simulink model "Copter_Plane_V10_sim_jy"  (R2021a)
settings: Solver=ode1  StartTime=0.0  StopTime=200  FixedStep=dt  RelTol=1e-3
undefined symbols (not defined in the file or in its folder): AC_Attitude, AC_PosControl, algo_accel_target_0, algo_accel_target_1, algo_accel_target_2, algo_arspeed, algo_attitude_target_euler_angle_0, algo_attitude_target_euler_angle_1, algo_attitude_target_euler_angle_2, algo_attitude_target_euler_rate_0, algo_attitude_target_euler_rate_1, algo_attitude_target_euler_rate_2, algo_climb_rate_cms, algo_curPathPoint_LLA_0, algo_curPathPoint_LLA_1, algo_curPosNED_0, algo_curPosNED_1, algo_curr_alt, algo_curr_pos_0, algo_curr_pos_1, algo_curr_vel_0, algo_curr_vel_1, algo_curr_vel_2, algo_current_loc_0, algo_current_loc_1, algo_curVelNED_0, algo_curVelNED_1, algo_flightControlMode, algo_flightTaskMode, algo_heightCmd_sl, algo_hgt_dem, algo_k_aileron, algo_k_elevator, algo_k_rudder, algo_k_throttle, algo_latAccDem, algo_limit_pos_up, algo_maxClimbSpeed, algo_mode, algo_nav_pitch_cd, algo_nav_roll, algo_pitch, algo_pitch_dem, algo_pitch_in, algo_pitch_target_pilot, algo_plane_mode, algo_pos_target_0, algo_pos_target_1, algo_pos_target_2, algo_prePathPoint_LLA_0, algo_prePathPoint_LLA_1, algo_pwm_out_1, algo_pwm_out_2, algo_pwm_out_3, algo_pwm_out_4, algo_rate_target_ang_vel_0, algo_rate_target_ang_vel_1, algo_rate_target_ang_vel_2, algo_remote_ct_st_pitch, algo_remote_ct_st_roll ... (+39)
libraries: aerolibasang x1, sharedtransform x1
(part 1 of 2)
settings Model: PauseTimes=6.8  Creator=a4327481  LastModifiedBy=a4327481
settings SolverCC: AlgebraicLoopSolver=TrustRegion
settings DebuggingCC: SFMachineParentedDataDiag=warning

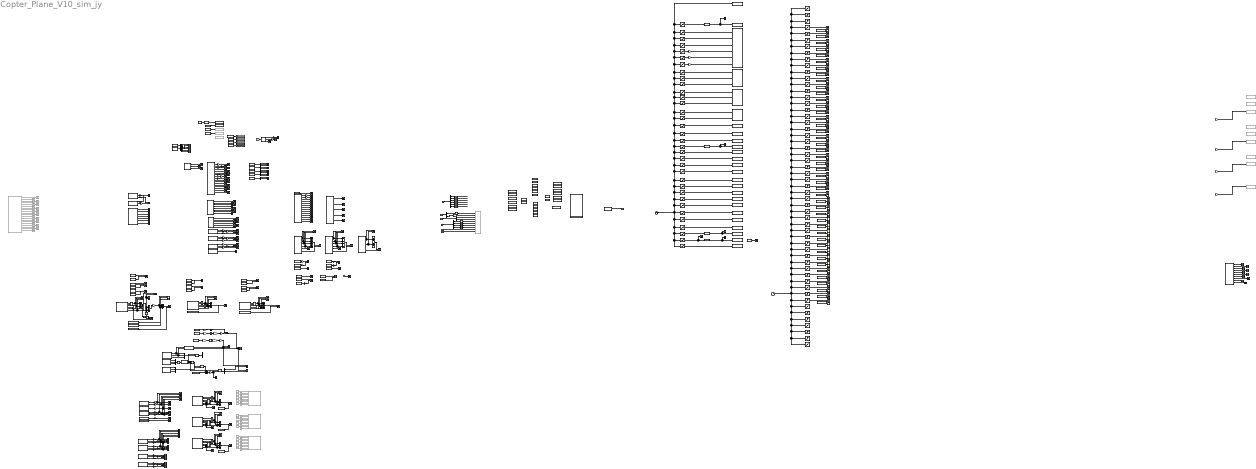
== system Copter_Plane_V10_sim_jy ==
  CTRL_wp : Inport
  PathModeOut : Inport  Port=2  OutDataTypeStr=Bus: BUS_TASK_PATH_OutParam
  TASK_COMMON_OutParam : Inport  Port=3  OutDataTypeStr=Bus: BUS_TASK_COMMON_OutParam
  NAVI2CONTROL : Inport  Port=4  OutDataTypeStr=Bus: BUS_TO_CONTROL
  EAS_Algo : Inport  Port=5  OutDataTypeStr=Bus: BUS_AIRSPEED
  IMU : Inport  Port=6  OutDataTypeStr=Bus: BUS_IMU
  AC_Attitude : DataStoreMemory  DataStoreName=AC_Attitude  ReadBeforeWriteMsg=warning  WriteAfterWriteMsg=warning  WriteAfterReadMsg=warning  InitialValue=AC_Attitude  ShowAdditionalParam=off  OutDataTypeStr=Bus: BUS_CTRL_AC_Attitude
  AC_PosControl : DataStoreMemory  DataStoreName=AC_PosControl  ReadBeforeWriteMsg=warning  WriteAfterWriteMsg=warning  WriteAfterReadMsg=warning  InitialValue=AC_PosControl  ShowAdditionalParam=off  OutDataTypeStr=Bus: BUS_CTRL_AC_PosControl
  AC_rate_pitch_pid : DataStoreMemory  DataStoreName=AC_rate_pitch_pid  ReadBeforeWriteMsg=warning  WriteAfterWriteMsg=warning  WriteAfterReadMsg=warning  InitialValue=AC_rate_pitch_pid  ShowAdditionalParam=off  OutDataTypeStr=Bus: BUS_CTRL_PID
  AC_rate_roll_pid : DataStoreMemory  DataStoreName=AC_rate_roll_pid  ReadBeforeWriteMsg=warning  WriteAfterWriteMsg=warning  WriteAfterReadMsg=warning  InitialValue=AC_rate_roll_pid  ShowAdditionalParam=off  OutDataTypeStr=Bus: BUS_CTRL_PID
  AC_rate_yaw_pid : DataStoreMemory  DataStoreName=AC_rate_yaw_pid  ReadBeforeWriteMsg=warning  WriteAfterWriteMsg=warning  WriteAfterReadMsg=warning  InitialValue=AC_rate_yaw_pid  ShowAdditionalParam=off  OutDataTypeStr=Bus: BUS_CTRL_PID
  AP_L1 : DataStoreMemory  DataStoreName=AP_L1  ReadBeforeWriteMsg=warning  WriteAfterWriteMsg=warning  WriteAfterReadMsg=warning  InitialValue=AP_L1  ShowAdditionalParam=off  OutDataTypeStr=Bus: BUS_CTRL_AP_L1
  AP_Motors : DataStoreMemory  DataStoreName=AP_Motors  ReadBeforeWriteMsg=warning  WriteAfterWriteMsg=warning  WriteAfterReadMsg=warning  InitialValue=AP_Motors  VectorParams1D=off  ShowAdditionalParam=off  OutDataTypeStr=Bus: BUS_CTRL_AP_Motors
  AP_TECS : DataStoreMemory  DataStoreName=AP_TECS  ReadBeforeWriteMsg=warning  WriteAfterWriteMsg=warning  WriteAfterReadMsg=warning  InitialValue=AP_TECS  ShowAdditionalParam=off  OutDataTypeStr=Bus: BUS_CTRL_AP_TECS
  AP_rate_pitch : DataStoreMemory  DataStoreName=AP_rate_pitch  ReadBeforeWriteMsg=warning  WriteAfterWriteMsg=warning  WriteAfterReadMsg=warning  InitialValue=AP_rate_pitch  ShowAdditionalParam=off  OutDataTypeStr=Bus: BUS_CTRL_AP_PID_pitch
  AP_rate_roll : DataStoreMemory  DataStoreName=AP_rate_roll  ReadBeforeWriteMsg=warning  WriteAfterWriteMsg=warning  WriteAfterReadMsg=warning  InitialValue=AP_rate_roll  ShowAdditionalParam=off  OutDataTypeStr=Bus: BUS_CTRL_AP_PID_roll
  AP_rate_yaw : DataStoreMemory  DataStoreName=AP_rate_yaw  ReadBeforeWriteMsg=warning  WriteAfterWriteMsg=warning  WriteAfterReadMsg=warning  InitialValue=AP_rate_yaw  ShowAdditionalParam=off  OutDataTypeStr=Bus: BUS_CTRL_AP_PID_yaw
  Add : Sum  Inputs=++++
  Add{4,6,10..13} (6 alike) : Sum  Inputs=+++
  Add14 : Sum  Inputs=++++
  Add{3,9,15..16} (4 alike) : Sum
  Bus Selector : BusSelector  OutputSignals=curVelNED,curLLA
  Bus Selector1 : BusSelector  OutputSignals=pitchd,rolld,yawd,alt
  Bus Selector2 : BusSelector  OutputSignals=gyro_x,gyro_y,gyro_z,accel_x,accel_y,accel_z
  Bus Selector3 : BusSelector  OutputSignals=airspeed_indicate,EAS2TAS_Algo
  Clock1 : Clock
  Clock2 : Clock
  Constant1 : Constant  Value=500/4500*0.95+0.05
  Constant10 : Constant  Value=500/4500*0.95+0.05
  Constant18 : Constant  Commented=on  Value=0.3
  Constant19 : Constant  Commented=on  Value=0.15
  Constant20 : Constant  Commented=on  Value=0.1
  Constant{21,26,33,38,43,48} (6 alike) : Constant  Commented=on  Value=0
  Constant22 : Constant  Commented=on  Value=0.25
  Constant{23..25,35..37,45..47} (9 alike) : Constant  Commented=on  Value=20
  Constant27 : Constant  Value=10  OutDataTypeStr=int16
  Constant28 : Constant  Commented=on
  Constant29 : Constant  Commented=on  Value=0.3
  Constant31 : Constant  Commented=on  Value=0.15
  Constant32 : Constant  Commented=on  Value=0.2
  Constant34 : Constant  Commented=on  Value=0.25
  Constant39 : Constant  Commented=on
  Constant40 : Constant  Commented=on  Value=0.3
  Constant41 : Constant  Commented=on  Value=0.15
  Constant42 : Constant  Commented=on  Value=0.1
  Constant44 : Constant  Commented=on  Value=0.25
  Constant49 : Constant  Commented=on
  Constant9 : Constant  Value=0.4
  Copter_Plane : DataStoreMemory  DataStoreName=Copter_Plane  ReadBeforeWriteMsg=warning  WriteAfterWriteMsg=warning  WriteAfterReadMsg=warning  InitialValue=Copter_Plane  VectorParams1D=off  ShowAdditionalParam=off  OutDataTypeStr=Bus: BUS_CTRL_Copter_Plane
  Curr_sate : DataStoreMemory  DataStoreName=Curr_sate  ReadBeforeWriteMsg=warning  WriteAfterWriteMsg=warning  WriteAfterReadMsg=warning  InitialValue=Curr_sate  VectorParams1D=off  ShowAdditionalParam=off  OutDataTypeStr=Bus: BUS_CTRL_Curr_sate
  Data Store Read : DataStoreRead  DataStoreName=SRV_Channel  IndexOptions=Index vector (dialog)  Indices=1  OutputSizes=1
  Data Store Read1 : DataStoreRead  DataStoreName=SINS  DataStoreElements=SINS.gyro_x#SINS.gyro_y#SINS.gyro_z#SINS.accel_x#SINS.accel_y#SINS.accel_z#SINS.roll#SINS.pitch#SINS.yaw#SINS.curr_vel(:,:)#SINS.curr_loc(:,:)#SINS.curr_alt#SINS.aspeed#SINS.EAS2TAS#SINS.groundspeed_vector(:,:)#SINS.curr_pos(:,:)#SINS.z_accel_meas  IndexOptions=Index vector (dialog)  Indices=1  OutputSizes=1
  Data Store Read10 : DataStoreRead  DataStoreName=AC_PosControl  DataStoreElements=AC_PosControl.vel_target(:,2)  IndexOptions=Index vector (dialog)  Indices=1  OutputSizes=1
  Data Store Read100 : DataStoreRead  DataStoreName=AP_rate_pitch  DataStoreElements=AP_rate_pitch.pid_info_P#AP_rate_pitch.pid_info_I#AP_rate_pitch.pid_info_D#AP_rate_pitch.pid_info_FF#AP_rate_pitch.pid_info_Dmod#AP_rate_pitch.last_out  IndexOptions=Index vector (dialog)  Indices=1  OutputSizes=1
  Data Store Read101 : DataStoreRead  DataStoreName=AP_rate_yaw  DataStoreElements=AP_rate_yaw.pid_info_I#AP_rate_yaw.pid_info_D#AP_rate_yaw.last_out  IndexOptions=Index vector (dialog)  Indices=1  OutputSizes=1
  Data Store Read105 : DataStoreRead  DataStoreName=AP_L1  DataStoreElements=AP_L1.L1_dist#AP_L1.last_Nu#AP_L1.latAccDem#AP_L1.nav_bearing#AP_L1.bearing_error  IndexOptions=Index vector (dialog)  Indices=1  OutputSizes=1
  Data Store Read107 : DataStoreRead  DataStoreName=AC_PosControl  DataStoreElements=AC_PosControl.accel_desired(:,:)  IndexOptions=Index vector (dialog)  Indices=1  OutputSizes=1
  Data Store Read108 : DataStoreRead  DataStoreName=AC_PosControl  DataStoreElements=AC_PosControl.accel_target(:,:)  IndexOptions=Index vector (dialog)  Indices=1  OutputSizes=1
  Data Store Read109 : DataStoreRead  DataStoreName=SINS  DataStoreElements=SINS.curr_vel(:,:)  IndexOptions=Index vector (dialog)  Indices=1  OutputSizes=1
  Data Store Read11 : DataStoreRead  DataStoreName=AC_PosControl  DataStoreElements=AC_PosControl.pos_target(:,2)  IndexOptions=Index vector (dialog)  Indices=1  OutputSizes=1
  Data Store Read112 : DataStoreRead  DataStoreName=AC_PosControl  DataStoreElements=AC_PosControl.vel_target(:,:)  IndexOptions=Index vector (dialog)  Indices=1  OutputSizes=1
  Data Store Read114 : DataStoreRead  DataStoreName=AC_PosControl  DataStoreElements=AC_PosControl.accel_target(:,3)  IndexOptions=Index vector (dialog)  Indices=1  OutputSizes=1
  Data Store Read116 : DataStoreRead  DataStoreName=SINS  DataStoreElements=SINS.z_accel_meas  IndexOptions=Index vector (dialog)  Indices=1  OutputSizes=1
  Data Store Read117 : DataStoreRead  DataStoreName=SINS  DataStoreElements=SINS.curr_vel(:,3)  IndexOptions=Index vector (dialog)  Indices=1  OutputSizes=1
  Data Store Read118 : DataStoreRead  DataStoreName=AC_PosControl  DataStoreElements=AC_PosControl.vel_desired(:,3)#AC_PosControl.vel_target(:,3)  IndexOptions=Index vector (dialog)  Indices=1  OutputSizes=1
  Data Store Read119 : DataStoreRead  DataStoreName=AC_PosControl  DataStoreElements=AC_PosControl.pos_target(:,3)  IndexOptions=Index vector (dialog)  Indices=1  OutputSizes=1
  Data Store Read12 : DataStoreRead  DataStoreName=AC_PosControl  DataStoreElements=AC_PosControl.pos_target(:,1)  IndexOptions=Index vector (dialog)  Indices=1  OutputSizes=1
  Data Store Read120 : DataStoreRead  DataStoreName=SINS  DataStoreElements=SINS.curr_alt  IndexOptions=Index vector (dialog)  Indices=1  OutputSizes=1
  Data Store Read123 : DataStoreRead  DataStoreName=AC_PosControl  DataStoreElements=AC_PosControl.vel_target(:,1)  IndexOptions=Index vector (dialog)  Indices=1  OutputSizes=1
  Data Store Read124 : DataStoreRead  DataStoreName=AC_PosControl  DataStoreElements=AC_PosControl.pos_target(:,1)  IndexOptions=Index vector (dialog)  Indices=1  OutputSizes=1
  Data Store Read125 : DataStoreRead  DataStoreName=SINS  DataStoreElements=SINS.curr_pos(:,1)  IndexOptions=Index vector (dialog)  Indices=1  OutputSizes=1
  Data Store Read13 : DataStoreRead  DataStoreName=AC_PosControl  DataStoreElements=AC_PosControl.pos_target(:,2)  IndexOptions=Index vector (dialog)  Indices=1  OutputSizes=1
  Data Store Read132 : DataStoreRead  DataStoreName=AP_Motors  DataStoreElements=AP_Motors.throttle_hover  IndexOptions=Index vector (dialog)  Indices=1  OutputSizes=1
  Data Store Read135 : DataStoreRead  DataStoreName=AP_Motors  DataStoreElements=AP_Motors.throttle_in  IndexOptions=Index vector (dialog)  Indices=1  OutputSizes=1
  Data Store Read137 : DataStoreRead  DataStoreName=AP_Motors  DataStoreElements=AP_Motors.angle_boost  IndexOptions=Index vector (dialog)  Indices=1  OutputSizes=1
  Data Store Read138 : DataStoreRead  DataStoreName=AC_Attitude  DataStoreElements=AC_Attitude.rate_target_ang_vel(:,1)#AC_Attitude.rate_target_ang_vel(:,2)#AC_Attitude.rate_target_ang_vel(:,3)  IndexOptions=Index vector (dialog)  Indices=1  OutputSizes=1
  Data Store Read139 : DataStoreRead  DataStoreName=SINS  DataStoreElements=SINS.curr_pos(:,2)  IndexOptions=Index vector (dialog)  Indices=1  OutputSizes=1
  Data Store Read14 : DataStoreRead  DataStoreName=SRV_Channel  DataStoreElements=SRV_Channel.k_rudder#SRV_Channel.k_aileron#SRV_Channel.k_elevator#SRV_Channel.k_throttle#SRV_Channel.k_flap#SRV_Channel.tail_tilt#SRV_Channel.pwm_tail#SRV_Channel.pwm_out(:,:)  IndexOptions=Index vector (dialog)  Indices=1  OutputSizes=1
  Data Store Read140 : DataStoreRead  DataStoreName=SINS  DataStoreElements=SINS.curr_vel(:,2)  IndexOptions=Index vector (dialog)  Indices=1  OutputSizes=1
  Data Store Read141 : DataStoreRead  DataStoreName=SINS  DataStoreElements=SINS.gyro_x#SINS.gyro_y#SINS.gyro_z  IndexOptions=Index vector (dialog)  Indices=1  OutputSizes=1
  Data Store Read142 : DataStoreRead  DataStoreName=SINS  DataStoreElements=SINS.roll#SINS.pitch#SINS.yaw  IndexOptions=Index vector (dialog)  Indices=1  OutputSizes=1
  Data Store Read144 : DataStoreRead  DataStoreName=SINS  DataStoreElements=SINS.curr_alt  IndexOptions=Index vector (dialog)  Indices=1  OutputSizes=1
  Data Store Read145 : DataStoreRead  DataStoreName=SINS  DataStoreElements=SINS.aspeed  IndexOptions=Index vector (dialog)  Indices=1  OutputSizes=1
  Data Store Read146 : DataStoreRead  DataStoreName=AP_TECS  DataStoreElements=AP_TECS.TAS_dem_adj  IndexOptions=Index vector (dialog)  Indices=1  OutputSizes=1
  Data Store Read147 : DataStoreRead  DataStoreName=SRV_Channel  DataStoreElements=SRV_Channel.k_throttle  IndexOptions=Index vector (dialog)  Indices=1  OutputSizes=1
  Data Store Read148 : DataStoreRead  DataStoreName=AC_Attitude  DataStoreElements=AC_Attitude.attitude_target_ang_vel(:,1)#AC_Attitude.attitude_target_ang_vel(:,2)#AC_Attitude.attitude_target_ang_vel(:,3)  IndexOptions=Index vector (dialog)  Indices=1  OutputSizes=1
  Data Store Read149 : DataStoreRead  DataStoreName=AC_Attitude  DataStoreElements=AC_Attitude.attitude_target_quat(:,:)  IndexOptions=Index vector (dialog)  Indices=1  OutputSizes=1
  Data Store Read15 : DataStoreRead  DataStoreName=AP_Motors  DataStoreElements=AP_Motors.yaw_in  IndexOptions=Index vector (dialog)  Indices=1  OutputSizes=1
  Data Store Read152 : DataStoreRead  DataStoreName=AC_Attitude  DataStoreElements=AC_Attitude.attitude_target_euler_rate(:,1)#AC_Attitude.attitude_target_euler_rate(:,2)#AC_Attitude.attitude_target_euler_rate(:,3)  IndexOptions=Index vector (dialog)  Indices=1  OutputSizes=1
  Data Store Read154 : DataStoreRead  Commented=on  DataStoreName=SlewLimiter  DataStoreElements=SlewLimiter.pos_event_stored#SlewLimiter.neg_event_stored#SlewLimiter.pos_event_index#SlewLimiter.neg_event_index#SlewLimiter.pos_event_ms(:,:)#SlewLimiter.neg_event_ms(:,:)#SlewLimiter.max_pos_slew_rate#SlewLimiter.max_neg_slew_rate#SlewLimiter.modifier_slew_rate#SlewLimiter.output_slew_rate#SlewLimiter.last_sample#SlewLimiter.slew_filter#SlewLimiter.N_EVENTS#SlewLimiter.max_pos_slew_event_ms#SlewLimiter.max_neg_slew_event_ms#SlewLimiter.MODIFIER_GAIN#SlewLimiter.WINDOW_MS#SlewLimiter.DERIVATIVE_CUTOFF_FREQ#SlewLimiter.slew_rate_max#SlewLimiter.slew_rate_tau  IndexOptions=Index vector (dialog)  Indices=1  OutputSizes=1
  Data Store Read16 : DataStoreRead  DataStoreName=AC_PosControl  DataStoreElements=AC_PosControl.pos_target(:,3)  IndexOptions=Index vector (dialog)  Indices=1  OutputSizes=1
  Data Store Read166 : DataStoreRead  DataStoreName=AC_PosControl  DataStoreElements=AC_PosControl.roll_target#AC_PosControl.pitch_target  IndexOptions=Index vector (dialog)  Indices=1  OutputSizes=1
  Data Store Read167 : DataStoreRead  DataStoreName=AC_Attitude  DataStoreElements=AC_Attitude.attitude_target_euler_angle(:,3)  IndexOptions=Index vector (dialog)  Indices=1  OutputSizes=1
  Data Store Read17 : DataStoreRead  DataStoreName=SINS  DataStoreElements=SINS.curr_pos(:,1)  IndexOptions=Index vector (dialog)  Indices=1  OutputSizes=1
  Data Store Read171 : DataStoreRead  DataStoreName=SINS  DataStoreElements=SINS.accel_x#SINS.accel_y#SINS.accel_z  IndexOptions=Index vector (dialog)  Indices=1  OutputSizes=1
  Data Store Read172 : DataStoreRead  DataStoreName=AC_PosControl  DataStoreElements=AC_PosControl.accel_target(:,1)#AC_PosControl.accel_target(:,2)#AC_PosControl.accel_target(:,3)  IndexOptions=Index vector (dialog)  Indices=1  OutputSizes=1
  Data Store Read174 : DataStoreRead  DataStoreName=SINS  DataStoreElements=SINS.roll#SINS.pitch#SINS.yaw  IndexOptions=Index vector (dialog)  Indices=1  OutputSizes=1
  Data Store Read18 : DataStoreRead  DataStoreName=plane_mode  IndexOptions=Index vector (dialog)  Indices=1  OutputSizes=1
  Data Store Read19 : DataStoreRead  DataStoreName=AP_Motors  DataStoreElements=AP_Motors.thrust_rpyt_out(:,:)#AP_Motors.throttle_filter#AP_Motors.roll_in#AP_Motors.pitch_in#AP_Motors.yaw_in#AP_Motors.throttle_in  IndexOptions=Index vector (dialog)  Indices=1  OutputSizes=1
  Data Store Read2 : DataStoreRead  DataStoreName=SRV_Channel  DataStoreElements=SRV_Channel.k_elevator  IndexOptions=Index vector (dialog)  Indices=1  OutputSizes=1
  Data Store Read20 : DataStoreRead  DataStoreName=SINS  DataStoreElements=SINS.curr_pos(:,2)  IndexOptions=Index vector (dialog)  Indices=1  OutputSizes=1
  Data Store Read21 : DataStoreRead  DataStoreName=Test_w  DataStoreElements=Test_w.roll_in#Test_w.pitch_in#Test_w.yaw_in#Test_w.throttle_in#Test_w.k_rudder#Test_w.k_elevator#Test_w.k_throttle#Test_w.k_aileron#Test_w.k_flap#Test_w.out  IndexOptions=Index vector (dialog)  Indices=1  OutputSizes=1
  Data Store Read22 : DataStoreRead  DataStoreName=Plane  DataStoreElements=Plane.nav_roll_cd#Plane.nav_pitch_cd  IndexOptions=Index vector (dialog)  Indices=1  OutputSizes=1
  Data Store Read23 : DataStoreRead  DataStoreName=SINS  DataStoreElements=SINS.roll#SINS.pitch#SINS.yaw  IndexOptions=Index vector (dialog)  Indices=1  OutputSizes=1
  Data Store Read24 : DataStoreRead  DataStoreName=AP_rate_pitch  DataStoreElements=AP_rate_pitch.pid_info_target#AP_rate_pitch.pid_info_actual#AP_rate_pitch.pid_info_error#AP_rate_pitch.pid_info_P#AP_rate_pitch.pid_info_I#AP_rate_pitch.pid_info_FF#AP_rate_pitch.pid_info_D  IndexOptions=Index vector (dialog)  Indices=1  OutputSizes=1
  Data Store Read25 : DataStoreRead  DataStoreName=PathModeOut_sl  DataStoreElements=PathModeOut_sl.flightControlMode  IndexOptions=Index vector (dialog)  Indices=1  OutputSizes=1
  Data Store Read26 : DataStoreRead  DataStoreName=Copter_Plane  DataStoreElements=Copter_Plane.roll_target_pilot#Copter_Plane.pitch_target_pilot#Copter_Plane.climb_rate_cms  IndexOptions=Index vector (dialog)  Indices=1  OutputSizes=1
  Data Store Read27 : DataStoreRead  DataStoreName=AC_PosControl  DataStoreElements=AC_PosControl.accel_target(:,1)  IndexOptions=Index vector (dialog)  Indices=1  OutputSizes=1
  Data Store Read28 : DataStoreRead  DataStoreName=AC_PosControl  DataStoreElements=AC_PosControl.accel_target(:,2)  IndexOptions=Index vector (dialog)  Indices=1  OutputSizes=1
  Data Store Read29 : DataStoreRead  DataStoreName=AC_PosControl  DataStoreElements=AC_PosControl.pid_vel_xy.kp#AC_PosControl.pid_vel_xy.error(:,2)#AC_PosControl.pid_vel_xy.kd#AC_PosControl.pid_vel_xy.derivative(:,2)#AC_PosControl.pid_vel_xy.integrator(:,2)  IndexOptions=Index vector (dialog)  Indices=1  OutputSizes=1
  Data Store Read3 : DataStoreRead  DataStoreName=AC_rate_pitch_pid  DataStoreElements=AC_rate_pitch_pid.kp#AC_rate_pitch_pid.error#AC_rate_pitch_pid.kd#AC_rate_pitch_pid.derivative#AC_rate_pitch_pid.Dmod#AC_rate_pitch_pid.integrator  IndexOptions=Index vector (dialog)  Indices=1  OutputSizes=1
  Data Store Read30 : DataStoreRead  DataStoreName=AC_PosControl  DataStoreElements=AC_PosControl.pid_vel_xy.kp#AC_PosControl.pid_vel_xy.error(:,1)#AC_PosControl.pid_vel_xy.kd#AC_PosControl.pid_vel_xy.derivative(:,1)#AC_PosControl.pid_vel_xy.integrator(:,1)  IndexOptions=Index vector (dialog)  Indices=1  OutputSizes=1
  Data Store Read31 : DataStoreRead  DataStoreName=AC_Attitude  DataStoreElements=AC_Attitude.attitude_target_euler_angle(:,:)  IndexOptions=Index vector (dialog)  Indices=1  OutputSizes=1
  Data Store Read32 : DataStoreRead  DataStoreName=AC_PosControl  DataStoreElements=AC_PosControl.vel_target(:,1)  IndexOptions=Index vector (dialog)  Indices=1  OutputSizes=1
  Data Store Read33 : DataStoreRead  DataStoreName=AC_PosControl  DataStoreElements=AC_PosControl.vel_target(:,2)  IndexOptions=Index vector (dialog)  Indices=1  OutputSizes=1
  Data Store Read34 : DataStoreRead  DataStoreName=AC_PosControl  DataStoreElements=AC_PosControl.vel_target(:,3)  IndexOptions=Index vector (dialog)  Indices=1  OutputSizes=1
  Data Store Read35 : DataStoreRead  DataStoreName=AC_PosControl  DataStoreElements=AC_PosControl.vel_desired(:,3)  IndexOptions=Index vector (dialog)  Indices=1  OutputSizes=1
  Data Store Read36 : DataStoreRead  DataStoreName=AC_PosControl  DataStoreElements=AC_PosControl.accel_target(:,1)  IndexOptions=Index vector (dialog)  Indices=1  OutputSizes=1
  Data Store Read37 : DataStoreRead  DataStoreName=AC_PosControl  DataStoreElements=AC_PosControl.accel_target(:,2)  IndexOptions=Index vector (dialog)  Indices=1  OutputSizes=1
  Data Store Read38 : DataStoreRead  DataStoreName=AC_PosControl  DataStoreElements=AC_PosControl.accel_target(:,3)  IndexOptions=Index vector (dialog)  Indices=1  OutputSizes=1
  Data Store Read39 : DataStoreRead  DataStoreName=SINS  DataStoreElements=SINS.z_accel_meas  IndexOptions=Index vector (dialog)  Indices=1  OutputSizes=1
  Data Store Read4 : DataStoreRead  DataStoreName=AP_Motors  DataStoreElements=AP_Motors.pitch_in  IndexOptions=Index vector (dialog)  Indices=1  OutputSizes=1
  Data Store Read40 : DataStoreRead  DataStoreName=Copter_Plane  DataStoreElements=Copter_Plane.climb_rate_cms  IndexOptions=Index vector (dialog)  Indices=1  OutputSizes=1
  Data Store Read41 : DataStoreRead  DataStoreName=AC_Attitude  DataStoreElements=AC_Attitude.attitude_target_euler_angle(:,1)  IndexOptions=Index vector (dialog)  Indices=1  OutputSizes=1
  Data Store Read42 : DataStoreRead  DataStoreName=AC_Attitude  DataStoreElements=AC_Attitude.attitude_target_euler_angle(:,2)  IndexOptions=Index vector (dialog)  Indices=1  OutputSizes=1
  Data Store Read43 : DataStoreRead  DataStoreName=AC_Attitude  DataStoreElements=AC_Attitude.attitude_target_euler_angle(:,3)  IndexOptions=Index vector (dialog)  Indices=1  OutputSizes=1
  Data Store Read44 : DataStoreRead  DataStoreName=AC_Attitude  DataStoreElements=AC_Attitude.attitude_target_euler_rate(:,1)  IndexOptions=Index vector (dialog)  Indices=1  OutputSizes=1
  Data Store Read45 : DataStoreRead  DataStoreName=AC_Attitude  DataStoreElements=AC_Attitude.attitude_target_euler_rate(:,2)  IndexOptions=Index vector (dialog)  Indices=1  OutputSizes=1
  Data Store Read46 : DataStoreRead  DataStoreName=AC_Attitude  DataStoreElements=AC_Attitude.attitude_target_euler_rate(:,3)  IndexOptions=Index vector (dialog)  Indices=1  OutputSizes=1
  Data Store Read47 : DataStoreRead  DataStoreName=AP_TECS  DataStoreElements=AP_TECS.hgt_dem_adj  IndexOptions=Index vector (dialog)  Indices=1  OutputSizes=1
  Data Store Read48 : DataStoreRead  DataStoreName=AC_Attitude  DataStoreElements=AC_Attitude.rate_target_ang_vel(:,1)  IndexOptions=Index vector (dialog)  Indices=1  OutputSizes=1
  Data Store Read49 : DataStoreRead  DataStoreName=Plane  DataStoreElements=Plane.nav_roll_cd  IndexOptions=Index vector (dialog)  Indices=1  OutputSizes=1
  Data Store Read5 : DataStoreRead  DataStoreName=AC_rate_roll_pid  DataStoreElements=AC_rate_roll_pid.kp#AC_rate_roll_pid.error#AC_rate_roll_pid.kd#AC_rate_roll_pid.derivative#AC_rate_roll_pid.Dmod#AC_rate_roll_pid.integrator  IndexOptions=Index vector (dialog)  Indices=1  OutputSizes=1
  Data Store Read50 : DataStoreRead  DataStoreName=AC_Attitude  DataStoreElements=AC_Attitude.rate_target_ang_vel(:,2)  IndexOptions=Index vector (dialog)  Indices=1  OutputSizes=1
  Data Store Read51 : DataStoreRead  DataStoreName=AC_Attitude  DataStoreElements=AC_Attitude.rate_target_ang_vel(:,3)  IndexOptions=Index vector (dialog)  Indices=1  OutputSizes=1
  Data Store Read52 : DataStoreRead  DataStoreName=AP_Motors  DataStoreElements=AP_Motors.roll_in  IndexOptions=Index vector (dialog)  Indices=1  OutputSizes=1
  Data Store Read53 : DataStoreRead  DataStoreName=AP_Motors  DataStoreElements=AP_Motors.pitch_in  IndexOptions=Index vector (dialog)  Indices=1  OutputSizes=1
  Data Store Read54 : DataStoreRead  DataStoreName=AP_Motors  DataStoreElements=AP_Motors.yaw_in  IndexOptions=Index vector (dialog)  Indices=1  OutputSizes=1
  Data Store Read55 : DataStoreRead  DataStoreName=AP_Motors  DataStoreElements=AP_Motors.throttle_in  IndexOptions=Index vector (dialog)  Indices=1  OutputSizes=1
  Data Store Read56 : DataStoreRead  DataStoreName=Copter_Plane  DataStoreElements=Copter_Plane.Mode  IndexOptions=Index vector (dialog)  Indices=1  OutputSizes=1
  Data Store Read57 : DataStoreRead  DataStoreName=AC_Attitude  DataStoreElements=AC_Attitude.attitude_target_euler_angle(:,1)#AC_Attitude.attitude_target_euler_angle(:,2)#AC_Attitude.attitude_target_euler_angle(:,3)  IndexOptions=Index vector (dialog)  Indices=1  OutputSizes=1
  Data Store Read58 : DataStoreRead  DataStoreName=AP_Motors  DataStoreElements=AP_Motors.throttle_filter  IndexOptions=Index vector (dialog)  Indices=1  OutputSizes=1
  Data Store Read59 : DataStoreRead  DataStoreName=Copter_Plane  DataStoreElements=Copter_Plane.weathervane_last_output  IndexOptions=Index vector (dialog)  Indices=1  OutputSizes=1
  Data Store Read6 : DataStoreRead  DataStoreName=AP_Motors  DataStoreElements=AP_Motors.roll_in  IndexOptions=Index vector (dialog)  Indices=1  OutputSizes=1
  Data Store Read60 : DataStoreRead  DataStoreName=PathModeOut_sl  DataStoreElements=PathModeOut_sl.flightTaskMode  IndexOptions=Index vector (dialog)  Indices=1  OutputSizes=1
  Data Store Read61 : DataStoreRead  DataStoreName=SRV_Channel  DataStoreElements=SRV_Channel.pwm_out(:,1)  IndexOptions=Index vector (dialog)  Indices=1  OutputSizes=1
  Data Store Read62 : DataStoreRead  DataStoreName=AC_Attitude  DataStoreElements=AC_Attitude.attitude_target_euler_rate(:,1)#AC_Attitude.attitude_target_euler_rate(:,2)#AC_Attitude.attitude_target_euler_rate(:,3)  IndexOptions=Index vector (dialog)  Indices=1  OutputSizes=1
  Data Store Read63 : DataStoreRead  DataStoreName=AC_Attitude  DataStoreElements=AC_Attitude.attitude_target_ang_vel(:,1)#AC_Attitude.attitude_target_ang_vel(:,2)#AC_Attitude.attitude_target_ang_vel(:,3)  IndexOptions=Index vector (dialog)  Indices=1  OutputSizes=1
  Data Store Read64 : DataStoreRead  DataStoreName=AP_Motors  DataStoreElements=AP_Motors.thrust_rpyt_out(:,:)  IndexOptions=Index vector (dialog)  Indices=1  OutputSizes=1
  Data Store Read65 : DataStoreRead  DataStoreName=SRV_Channel  DataStoreElements=SRV_Channel.pwm_out(:,2)  IndexOptions=Index vector (dialog)  Indices=1  OutputSizes=1
  Data Store Read66 : DataStoreRead  DataStoreName=SRV_Channel  DataStoreElements=SRV_Channel.pwm_out(:,3)  IndexOptions=Index vector (dialog)  Indices=1  OutputSizes=1
  Data Store Read67 : DataStoreRead  DataStoreName=SRV_Channel  DataStoreElements=SRV_Channel.pwm_out(:,4)  IndexOptions=Index vector (dialog)  Indices=1  OutputSizes=1
  Data Store Read68 : DataStoreRead  DataStoreName=AC_PosControl  DataStoreElements=AC_PosControl.pos_target(:,:)  IndexOptions=Index vector (dialog)  Indices=1  OutputSizes=1
  Data Store Read69 : DataStoreRead  DataStoreName=SRV_Channel  DataStoreElements=SRV_Channel.tail_tilt  IndexOptions=Index vector (dialog)  Indices=1  OutputSizes=1
  Data Store Read7 : DataStoreRead  DataStoreName=SRV_Channel  DataStoreElements=SRV_Channel.k_aileron  IndexOptions=Index vector (dialog)  Indices=1  OutputSizes=1
  Data Store Read70 : DataStoreRead  DataStoreName=Plane  DataStoreElements=Plane.nav_pitch_cd  IndexOptions=Index vector (dialog)  Indices=1  OutputSizes=1
  Data Store Read71 : DataStoreRead  DataStoreName=AC_PosControl  DataStoreElements=AC_PosControl.vel_desired(:,:)  IndexOptions=Index vector (dialog)  Indices=1  OutputSizes=1
  Data Store Read72 : DataStoreRead  DataStoreName=SINS  DataStoreElements=SINS.aspeed  IndexOptions=Index vector (dialog)  Indices=1  OutputSizes=1
  Data Store Read73 : DataStoreRead  DataStoreName=Plane  DataStoreElements=Plane.nav_pitch_cd  IndexOptions=Index vector (dialog)  Indices=1  OutputSizes=1
  Data Store Read74 : DataStoreRead  DataStoreName=AC_PosControl  DataStoreElements=AC_PosControl.vel_target(:,:)  IndexOptions=Index vector (dialog)  Indices=1  OutputSizes=1
  Data Store Read75 : DataStoreRead  DataStoreName=SINS  DataStoreElements=SINS.roll  IndexOptions=Index vector (dialog)  Indices=1  OutputSizes=1
  Data Store Read76 : DataStoreRead  DataStoreName=AC_PosControl  DataStoreElements=AC_PosControl.pitch_target  IndexOptions=Index vector (dialog)  Indices=1  OutputSizes=1
  Data Store Read77 : DataStoreRead  DataStoreName=Plane  DataStoreElements=Plane.nav_roll_cd  IndexOptions=Index vector (dialog)  Indices=1  OutputSizes=1
  Data Store Read78 : DataStoreRead  DataStoreName=AP_TECS  DataStoreElements=AP_TECS.pitch_dem  IndexOptions=Index vector (dialog)  Indices=1  OutputSizes=1
  Data Store Read79 : DataStoreRead  DataStoreName=AP_TECS  DataStoreElements=AP_TECS.throttle_dem  IndexOptions=Index vector (dialog)  Indices=1  OutputSizes=1
  Data Store Read8 : DataStoreRead  DataStoreName=AC_PosControl  DataStoreElements=AC_PosControl.pid_accel_z.kp#AC_PosControl.pid_accel_z.error#AC_PosControl.pid_accel_z.kd#AC_PosControl.pid_accel_z.derivative#AC_PosControl.pid_accel_z.Dmod#AC_PosControl.pid_accel_z.integrator  IndexOptions=Index vector (dialog)  Indices=1  OutputSizes=1
  Data Store Read80 : DataStoreRead  DataStoreName=AP_L1  DataStoreElements=AP_L1.latAccDem  IndexOptions=Index vector (dialog)  Indices=1  OutputSizes=1
  Data Store Read81 : DataStoreRead  DataStoreName=SRV_Channel  DataStoreElements=SRV_Channel.k_rudder  IndexOptions=Index vector (dialog)  Indices=1  OutputSizes=1
  Data Store Read82 : DataStoreRead  DataStoreName=SINS  DataStoreElements=SINS.pitch  IndexOptions=Index vector (dialog)  Indices=1  OutputSizes=1
  Data Store Read83 : DataStoreRead  DataStoreName=SRV_Channel  DataStoreElements=SRV_Channel.k_aileron  IndexOptions=Index vector (dialog)  Indices=1  OutputSizes=1
  Data Store Read84 : DataStoreRead  DataStoreName=SRV_Channel  DataStoreElements=SRV_Channel.k_elevator  IndexOptions=Index vector (dialog)  Indices=1  OutputSizes=1
  Data Store Read85 : DataStoreRead  DataStoreName=SRV_Channel  DataStoreElements=SRV_Channel.k_throttle  IndexOptions=Index vector (dialog)  Indices=1  OutputSizes=1
  Data Store Read86 : DataStoreRead  DataStoreName=Curr_sate  DataStoreElements=Curr_sate.PathModeOut.flightTaskMode  IndexOptions=Index vector (dialog)  Indices=1  OutputSizes=1
  Data Store Read9 : DataStoreRead  DataStoreName=AC_rate_yaw_pid  DataStoreElements=AC_rate_yaw_pid.kp#AC_rate_yaw_pid.error#AC_rate_yaw_pid.kd#AC_rate_yaw_pid.derivative#AC_rate_yaw_pid.Dmod#AC_rate_yaw_pid.integrator  IndexOptions=Index vector (dialog)  Indices=1  OutputSizes=1
  Data Store Read90 : DataStoreRead  DataStoreName=SINS  DataStoreElements=SINS.curr_vel(:,1)  IndexOptions=Index vector (dialog)  Indices=1  OutputSizes=1
  Data Store Read91 : DataStoreRead  DataStoreName=AC_PosControl  DataStoreElements=AC_PosControl.roll_target  IndexOptions=Index vector (dialog)  Indices=1  OutputSizes=1
  Data Store Read92 : DataStoreRead  DataStoreName=AC_PosControl  DataStoreElements=AC_PosControl.pitch_target  IndexOptions=Index vector (dialog)  Indices=1  OutputSizes=1
  Data Store Read97 : DataStoreRead  DataStoreName=AP_TECS  DataStoreElements=AP_TECS.PITCHmaxf#AP_TECS.PITCHminf#AP_TECS.TAS_dem#AP_TECS.TAS_dem_adj#AP_TECS.TAS_rate_dem#AP_TECS.hgt_dem_adj#AP_TECS.hgt_rate_dem#AP_TECS.TAS_state#AP_TECS.climb_rate#AP_TECS.vel_dot#AP_TECS.throttle_dem#AP_TECS.integTHR_state#AP_TECS.ff_throttle#AP_TECS.pitch_dem  IndexOptions=Index vector (dialog)  Indices=1  OutputSizes=1
  Data Store Read98 : DataStoreRead  DataStoreName=Plane  DataStoreElements=Plane.scaling_speed  IndexOptions=Index vector (dialog)  Indices=1  OutputSizes=1
  Data Store Read99 : DataStoreRead  DataStoreName=AP_rate_roll  DataStoreElements=AP_rate_roll.pid_info_P#AP_rate_roll.pid_info_I#AP_rate_roll.pid_info_D#AP_rate_roll.pid_info_FF#AP_rate_roll.pid_info_Dmod#AP_rate_roll.last_out  IndexOptions=Index vector (dialog)  Indices=1  OutputSizes=1
  Data Store Write1 : DataStoreWrite  Commented=on  DataStoreName=AC_rate_roll_pid  DataStoreElements=AC_rate_roll_pid.kp#AC_rate_roll_pid.ki#AC_rate_roll_pid.kd#AC_rate_roll_pid.kff#AC_rate_roll_pid.kimax#AC_rate_roll_pid.filt_T_hz#AC_rate_roll_pid.filt_E_hz#AC_rate_roll_pid.filt_D_hz#AC_rate_roll_pid.slew_rate_max#AC_rate_roll_pid.slew_rate_tau  IndexOptions=Index vector (dialog)  Indices=1  OutputSizes=1
  Data Store Write11 : DataStoreWrite  DataStoreName=Curr_sate  DataStoreElements=Curr_sate.EAS2TAS_Algo  IndexOptions=Index vector (dialog)  Indices=1  OutputSizes=1
  Data Store Write12 : DataStoreWrite  DataStoreName=algo_remote_ct_st  DataStoreElements=algo_remote_ct_st.throttle  IndexOptions=Index vector (dialog)  Indices=1  OutputSizes=1
  Data Store Write13 : DataStoreWrite  DataStoreName=Curr_sate  DataStoreElements=Curr_sate.gyro_x#Curr_sate.gyro_y#Curr_sate.gyro_z#Curr_sate.accel_x#Curr_sate.accel_y#Curr_sate.accel_z  IndexOptions=Index vector (dialog)  Indices=1  OutputSizes=1
  Data Store Write14 : DataStoreWrite  Commented=on  DataStoreName=algo_remote_ct_st  DataStoreElements=algo_remote_ct_st.roll  IndexOptions=Index vector (dialog)  Indices=1  OutputSizes=1
  Data Store Write15 : DataStoreWrite  Commented=on  DataStoreName=algo_remote_ct_st  DataStoreElements=algo_remote_ct_st.tail_throttle_pwm  IndexOptions=Index vector (dialog)  Indices=1  OutputSizes=1
  Data Store Write16 : DataStoreWrite  Commented=on  DataStoreName=AC_rate_yaw_pid  DataStoreElements=AC_rate_yaw_pid.kp#AC_rate_yaw_pid.ki#AC_rate_yaw_pid.kd#AC_rate_yaw_pid.kff#AC_rate_yaw_pid.kimax#AC_rate_yaw_pid.filt_T_hz#AC_rate_yaw_pid.filt_E_hz#AC_rate_yaw_pid.filt_D_hz#AC_rate_yaw_pid.slew_rate_max#AC_rate_yaw_pid.slew_rate_tau  IndexOptions=Index vector (dialog)  Indices=1  OutputSizes=1
  Data Store Write18 : DataStoreWrite  Commented=on  DataStoreName=Copter_Plane  DataStoreElements=Copter_Plane.hgt_dem_cm  IndexOptions=Index vector (dialog)  Indices=1  OutputSizes=1
  Data Store Write2 : DataStoreWrite  Commented=on  DataStoreName=Curr_sate  DataStoreElements=Curr_sate.EAS_Algo#Curr_sate.EAS2TAS_Algo#Curr_sate.curVelNED(:,:)#Curr_sate.curLLA(:,:)#Curr_sate.pitchd#Curr_sate.rolld#Curr_sate.yawd#Curr_sate.NAV_alt#Curr_sate.PathModeOut#Curr_sate.wp_in(:,:)  IndexOptions=Index vector (dialog)  Indices=1  OutputSizes=1
  Data Store Write20 : DataStoreWrite  DataStoreName=Curr_sate  DataStoreElements=Curr_sate.PathModeOut.heightCmd  IndexOptions=Index vector (dialog)  Indices=1  OutputSizes=1
  Data Store Write21 : DataStoreWrite  DataStoreName=Curr_sate  DataStoreElements=Curr_sate.PathModeOut.flightTaskMode  IndexOptions=Index vector (dialog)  Indices=1  OutputSizes=1
  Data Store Write22 : DataStoreWrite  DataStoreName=Curr_sate  DataStoreElements=Curr_sate.PathModeOut.maxClimbSpeed  IndexOptions=Index vector (dialog)  Indices=1  OutputSizes=1
  Data Store Write23 : DataStoreWrite  DataStoreName=Curr_sate  DataStoreElements=Curr_sate.PathModeOut.turnCenterLL(:,1)  IndexOptions=Index vector (dialog)  Indices=1  OutputSizes=1
  Data Store Write24 : DataStoreWrite  DataStoreName=Curr_sate  DataStoreElements=Curr_sate.PathModeOut.turnCenterLL(:,2)  IndexOptions=Index vector (dialog)  Indices=1  OutputSizes=1
  Data Store Write25 : DataStoreWrite  DataStoreName=Curr_sate  DataStoreElements=Curr_sate.PathModeOut.prePathPoint_LLA(:,1)  IndexOptions=Index vector (dialog)  Indices=1  OutputSizes=1
  Data Store Write26 : DataStoreWrite  DataStoreName=Curr_sate  DataStoreElements=Curr_sate.PathModeOut.prePathPoint_LLA(:,2)  IndexOptions=Index vector (dialog)  Indices=1  OutputSizes=1
  Data Store Write28 : DataStoreWrite  DataStoreName=Curr_sate  DataStoreElements=Curr_sate.curVelNED(:,1)#Curr_sate.curVelNED(:,2)#Curr_sate.curVelNED(:,3)  IndexOptions=Index vector (dialog)  Indices=1  OutputSizes=1
  Data Store Write29 : DataStoreWrite  DataStoreName=Curr_sate  DataStoreElements=Curr_sate.NAV_alt  IndexOptions=Index vector (dialog)  Indices=1  OutputSizes=1
  Data Store Write3 : DataStoreWrite  Commented=on  DataStoreName=AC_rate_pitch_pid  DataStoreElements=AC_rate_pitch_pid.kp#AC_rate_pitch_pid.ki#AC_rate_pitch_pid.kd#AC_rate_pitch_pid.kff#AC_rate_pitch_pid.kimax#AC_rate_pitch_pid.filt_T_hz#AC_rate_pitch_pid.filt_E_hz#AC_rate_pitch_pid.filt_D_hz#AC_rate_pitch_pid.slew_rate_max#AC_rate_pitch_pid.slew_rate_tau  IndexOptions=Index vector (dialog)  Indices=1  OutputSizes=1
  Data Store Write30 : DataStoreWrite  DataStoreName=Curr_sate  DataStoreElements=Curr_sate.PathModeOut.curPathPoint_LLA(:,1)  IndexOptions=Index vector (dialog)  Indices=1  OutputSizes=1
  Data Store Write31 : DataStoreWrite  DataStoreName=Curr_sate  DataStoreElements=Curr_sate.PathModeOut.curPathPoint_LLA(:,2)  IndexOptions=Index vector (dialog)  Indices=1  OutputSizes=1
  Data Store Write32 : DataStoreWrite  DataStoreName=Curr_sate  DataStoreElements=Curr_sate.PathModeOut.rollCmd  IndexOptions=Index vector (dialog)  Indices=1  OutputSizes=1
  Data Store Write33 : DataStoreWrite  Commented=on  DataStoreName=AC_PosControl  DataStoreElements=AC_PosControl.pos_target(:,3)  IndexOptions=Index vector (dialog)  Indices=1  OutputSizes=1
  Data Store Write34 : DataStoreWrite  Commented=on  DataStoreName=AC_PosControl  DataStoreElements=AC_PosControl.vel_desired(:,3)  IndexOptions=Index vector (dialog)  Indices=1  OutputSizes=1
  Data Store Write35 : DataStoreWrite  DataStoreName=algo_remote_ct_st  DataStoreElements=algo_remote_ct_st.Mode  IndexOptions=Index vector (dialog)  Indices=1  OutputSizes=1
  Data Store Write37 : DataStoreWrite  Commented=on  DataStoreName=Copter_Plane  DataStoreElements=Copter_Plane.climb_rate_cms  IndexOptions=Index vector (dialog)  Indices=1  OutputSizes=1
  Data Store Write38 : DataStoreWrite  DataStoreName=plane_mode  IndexOptions=Index vector (dialog)  Indices=1  OutputSizes=1
  Data Store Write39 : DataStoreWrite  DataStoreName=Curr_sate  DataStoreElements=Curr_sate.PathModeOut.flightControlMode  IndexOptions=Index vector (dialog)  Indices=1  OutputSizes=1
  Data Store Write4 : DataStoreWrite  Commented=on  DataStoreName=algo_remote_ct_st  DataStoreElements=algo_remote_ct_st.pitch  IndexOptions=Index vector (dialog)  Indices=1  OutputSizes=1
  Data Store Write40 : DataStoreWrite  DataStoreName=algo_remote_ct_st  DataStoreElements=algo_remote_ct_st.Mode  IndexOptions=Index vector (dialog)  Indices=1  OutputSizes=1
  Data Store Write41 : DataStoreWrite  Commented=on  DataStoreName=AP_TECS  DataStoreElements=AP_TECS.throttle_dem  IndexOptions=Index vector (dialog)  Indices=1  OutputSizes=1
  Data Store Write47 : DataStoreWrite  DataStoreName=algo_remote_ct_st  DataStoreElements=algo_remote_ct_st.pitch  IndexOptions=Index vector (dialog)  Indices=1  OutputSizes=1
  Data Store Write5 : DataStoreWrite  DataStoreName=systime  IndexOptions=Index vector (dialog)  Indices=1  OutputSizes=1
  Data Store Write52 : DataStoreWrite  Commented=on  DataStoreName=SINS  DataStoreElements=SINS.groundspeed_vector(:,1)  IndexOptions=Index vector (dialog)  Indices=1  OutputSizes=1
  Data Store Write53 : DataStoreWrite  DataStoreName=algo_remote_ct_st  DataStoreElements=algo_remote_ct_st.throttle  IndexOptions=Index vector (dialog)  Indices=1  OutputSizes=1
  Data Store Write58 : DataStoreWrite  DataStoreName=algo_remote_ct_st  DataStoreElements=algo_remote_ct_st.yaw  IndexOptions=Index vector (dialog)  Indices=1  OutputSizes=1
  Data Store Write60 : DataStoreWrite  Commented=on  DataStoreName=SINS  DataStoreElements=SINS.groundspeed_vector(:,2)  IndexOptions=Index vector (dialog)  Indices=1  OutputSizes=1
  Data Store Write63 : DataStoreWrite  DataStoreName=algo_remote_ct_st  DataStoreElements=algo_remote_ct_st.roll  IndexOptions=Index vector (dialog)  Indices=1  OutputSizes=1
  Data Store Write64 : DataStoreWrite  Commented=on  DataStoreName=SRV_Channel  DataStoreElements=SRV_Channel.tail_tilt  IndexOptions=Index vector (dialog)  Indices=1  OutputSizes=1
  Data Store Write66 : DataStoreWrite  Commented=on  DataStoreName=Plane  DataStoreElements=Plane.nav_pitch_cd  IndexOptions=Index vector (dialog)  Indices=1  OutputSizes=1
  Data Store Write7 : DataStoreWrite  DataStoreName=Curr_sate  DataStoreElements=Curr_sate.rolld#Curr_sate.pitchd#Curr_sate.yawd  IndexOptions=Index vector (dialog)  Indices=1  OutputSizes=1
  Data Store Write8 : DataStoreWrite  DataStoreName=Curr_sate  DataStoreElements=Curr_sate.curLLA(:,1)#Curr_sate.curLLA(:,2)  IndexOptions=Index vector (dialog)  Indices=1  OutputSizes=1
  Data Store Write9 : DataStoreWrite  DataStoreName=Curr_sate  DataStoreElements=Curr_sate.EAS_Algo  IndexOptions=Index vector (dialog)  Indices=1  OutputSizes=1
  Data Type Conversion{,1..11} (12 alike) : DataTypeConversion
  Data Type Conversion14 : DataTypeConversion  OutDataTypeStr=Enum: ENUM_Mode  RndMeth=Ceiling
  Data Type Conversion15 : DataTypeConversion  OutDataTypeStr=Enum: ENUM_FlightTaskMode  RndMeth=Ceiling
  Data Type Conversion16 : DataTypeConversion  OutDataTypeStr=Enum: ENUM_plane_mode  RndMeth=Ceiling  LockScale=on
  Data Type Conversion17 : DataTypeConversion  OutDataTypeStr=Enum: ENUM_FlightControlMode  RndMeth=Ceiling
  Data Type Conversion18 : DataTypeConversion  OutDataTypeStr=Enum: ENUM_Mode  RndMeth=Ceiling
  Demux{3..4,9,12..13,21..22,24..25} (9 alike) : Demux  Outputs=3
  Derivative : Derivative
  Derivative3 : Derivative
  Display{1,5..7} (4 alike) : Display
  Divide1 : Product  Inputs=/*
  Divide{6..11} (6 alike) : Product  Inputs=***
  Divide{4..5,12..16} (7 alike) : Product  Inputs=**
  EAS2TAS_Algo : Lookup_n-D  NumberOfTableDimensions=1  BreakpointsForDimension1=time_arspeed  Table=EAS2TAS_Algo  InternalRulePriority=Speed  RndMeth=Simplest  InputSameDT=on
  EAS_Algo1 : Lookup_n-D  NumberOfTableDimensions=1  BreakpointsForDimension1=time_arspeed  Table=EAS_Algo  InternalRulePriority=Speed  RndMeth=Simplest  InputSameDT=on
  GRAVITY_MSS1 : DataStoreMemory  DataStoreName=GRAVITY_MSS  ReadBeforeWriteMsg=warning  WriteAfterWriteMsg=warning  WriteAfterReadMsg=warning  InitialValue=GRAVITY_MSS  VectorParams1D=off  ShowAdditionalParam=off  OutDataTypeStr=double
  Gain{9..10,17,19,21} (5 alike) : Gain  Gain=0.01
  Gain{11..13,15..16,22,30..37,43,48..49,51,53..55,59..64,66..68,71..73,75,80..85} (40 alike) : Gain  Gain=HD
  Gain{50,70,137,147..148,164} (6 alike) : Gain  Gain=100
  Gain18 : Gain  Gain=1/100/HD
  Gain20 : Gain  Gain=1/100/HD
  Gain23 : Gain  Gain=GRAVITY_MSS
  Gain24 : Gain  Gain=-100
  Gain25 : Gain  Gain=1/100/HD
  Gain27 : Gain  Gain=GRAVITY_MSS
  Gain41 : Gain  Gain=1/HD
  Gain65 : Gain  Gain=0.001
  Gain86 : Gain  Gain=1/100
  Gain87 : Gain  Gain=1/100
  Gain91 : Gain  Gain=1/HD
  Gain92 : Gain  Gain=1/HD
  HD1 : DataStoreMemory  DataStoreName=HD  ReadBeforeWriteMsg=warning  WriteAfterWriteMsg=warning  WriteAfterReadMsg=warning  InitialValue=HD  ShowAdditionalParam=off  OutDataTypeStr=double
  "Incidence, Sideslip & Airspeed3" : aerolibasang/Incidence, Sideslip, & Airspeed
  LOCATION_SCALING_FACTOR1 : DataStoreMemory  DataStoreName=LOCATION_SCALING_FACTOR  ReadBeforeWriteMsg=warning  WriteAfterWriteMsg=warning  WriteAfterReadMsg=warning  InitialValue=LOCATION_SCALING_FACTOR  VectorParams1D=off  ShowAdditionalParam=off  OutDataTypeStr=double
  LOCATION_SCALING_FACTOR_INV : DataStoreMemory  DataStoreName=LOCATION_SCALING_FACTOR_INV  ReadBeforeWriteMsg=warning  WriteAfterWriteMsg=warning  WriteAfterReadMsg=warning  InitialValue=LOCATION_SCALING_FACTOR_INV  VectorParams1D=off  ShowAdditionalParam=off  OutDataTypeStr=double
  MATLAB Function17 : MATLAB Function  TreatAsAtomicUnit=on
  Mux10 : Mux  Inputs=3
  Mux2 : Mux  Inputs=2
  Mux3 : Mux  Inputs=3
  Mux7 : Mux  Inputs=3
  PathModeOut1 : DataStoreMemory  DataStoreName=PathModeOut_sl  ReadBeforeWriteMsg=warning  WriteAfterWriteMsg=warning  WriteAfterReadMsg=warning  InitialValue=PathModeOut_sl  VectorParams1D=off  ShowAdditionalParam=off  OutDataTypeStr=Bus: BUS_TASK_PATH_OutParam
  Plane : DataStoreMemory  DataStoreName=Plane  ReadBeforeWriteMsg=warning  WriteAfterWriteMsg=warning  WriteAfterReadMsg=warning  InitialValue=Plane  ShowAdditionalParam=off  OutDataTypeStr=Bus: BUS_CTRL_Plane
  Rotation Angles to Direction Cosine Matrix1 : sharedtransform/Rotation Angles to Direction Cosine Matrix  rotationOrder=ZYX  aMode=aMode
      settings: SourceProductBaseCode=AE,PW,DR,MT,UV,VE
  SINS : DataStoreMemory  DataStoreName=SINS  ReadBeforeWriteMsg=warning  WriteAfterWriteMsg=warning  WriteAfterReadMsg=warning  InitialValue=SINS  VectorParams1D=off  ShowAdditionalParam=off  OutDataTypeStr=Bus: BUS_CTRL_SINS
  SRV_Channel : DataStoreMemory  DataStoreName=SRV_Channel  ReadBeforeWriteMsg=warning  WriteAfterWriteMsg=warning  WriteAfterReadMsg=warning  InitialValue=SRV_Channel  ShowAdditionalParam=off  OutDataTypeStr=Bus: BUS_CTRL_SRV_Channel
  Scope{1,3..4,15..24,26..27,29..39,65..68,71,79,82,86,89..95,97,99..102,104,107..109,111..112,115..116,119..120,123,125,129..133,136,141,143..144,146,152,175,177..178,180..182,184..185,189..197,210..215,217..225,227,231..236,240..248,273..275} (120 alike) : Scope
  Scope{2,5,7,10,53,156,159,161,164..165,171,173,249} (13 alike) : Scope  NumInputPorts=3
  Scope{6,8..9,11..14,25,28,40..52,54..64,69..70,72..78,80..81,83..85,87..88,96,98,149,153,166..169,172,174,179,183,186..187,198..203,206..209,216,226,228..230,239,250..252} (82 alike) : Scope  NumInputPorts=2
  Scope237 : Scope  NumInputPorts=4
  Scope238 : Scope  NumInputPorts=4
  Scope{253..272} (20 alike) : Scope  Commented=on
  Selector2 : Selector  InputPortWidth=3  IndexOptions=Index vector (dialog)  Indices=[3 2 1]  OutputSizes=1
  SlewLimiter : DataStoreMemory  DataStoreName=SlewLimiter  ReadBeforeWriteMsg=warning  WriteAfterWriteMsg=warning  WriteAfterReadMsg=warning  InitialValue=SlewLimiter  VectorParams1D=off  ShowAdditionalParam=off  OutDataTypeStr=Bus: BUS_CTRL_SlewLimiter
  Tan : Trigonometry  Operator=tan
  Tan1 : Trigonometry  Operator=tan
  Tan2 : Trigonometry  Operator=cos
  Test_w : DataStoreMemory  DataStoreName=Test_w  ReadBeforeWriteMsg=warning  WriteAfterWriteMsg=warning  WriteAfterReadMsg=warning  InitialValue=Test_w  ShowAdditionalParam=off  OutDataTypeStr=Bus: BUS_CTRL_Test_w
  Transpose3 : Math  Operator=transpose  SignedPower=on  SaturateOnIntegerOverflow=on
  algo_accel_target_0 : Lookup_n-D  NumberOfTableDimensions=1  BreakpointsForDimension1=time_algo  Table=algo_accel_target_0  InternalRulePriority=Speed  RndMeth=Simplest  InputSameDT=on
  algo_accel_target_1 : Lookup_n-D  NumberOfTableDimensions=1  BreakpointsForDimension1=time_algo  Table=algo_accel_target_1  InternalRulePriority=Speed  RndMeth=Simplest  InputSameDT=on
  algo_accel_target_2 : Lookup_n-D  NumberOfTableDimensions=1  BreakpointsForDimension1=time_algo  Table=algo_accel_target_2  InternalRulePriority=Speed  RndMeth=Simplest  InputSameDT=on
  algo_arspeed : Lookup_n-D  NumberOfTableDimensions=1  BreakpointsForDimension1=time_algo  Table=algo_arspeed  InternalRulePriority=Speed  RndMeth=Simplest  InputSameDT=on
  algo_attitude_target_euler_angle_0 : Lookup_n-D  NumberOfTableDimensions=1  BreakpointsForDimension1=time_algo  Table=algo_attitude_target_euler_angle_0  InternalRulePriority=Speed  RndMeth=Simplest  InputSameDT=on
  algo_attitude_target_euler_angle_1 : Lookup_n-D  NumberOfTableDimensions=1  BreakpointsForDimension1=time_algo  Table=algo_attitude_target_euler_angle_1  InternalRulePriority=Speed  RndMeth=Simplest  InputSameDT=on
  algo_attitude_target_euler_angle_2 : Lookup_n-D  NumberOfTableDimensions=1  BreakpointsForDimension1=time_algo  Table=algo_attitude_target_euler_angle_2  InternalRulePriority=Speed  RndMeth=Simplest  InputSameDT=on
  algo_attitude_target_euler_rate_0 : Lookup_n-D  NumberOfTableDimensions=1  BreakpointsForDimension1=time_algo  Table=algo_attitude_target_euler_rate_0  InternalRulePriority=Speed  RndMeth=Simplest  InputSameDT=on
  algo_attitude_target_euler_rate_1 : Lookup_n-D  NumberOfTableDimensions=1  BreakpointsForDimension1=time_algo  Table=algo_attitude_target_euler_rate_1  InternalRulePriority=Speed  RndMeth=Simplest  InputSameDT=on
  algo_attitude_target_euler_rate_2 : Lookup_n-D  NumberOfTableDimensions=1  BreakpointsForDimension1=time_algo  Table=algo_attitude_target_euler_rate_2  InternalRulePriority=Speed  RndMeth=Simplest  InputSameDT=on
  algo_climb_rate_cms : Lookup_n-D  NumberOfTableDimensions=1  BreakpointsForDimension1=time_algo  Table=algo_climb_rate_cms  InternalRulePriority=Speed  RndMeth=Simplest  InputSameDT=on
  algo_curPathPoint_LLA_0 : Lookup_n-D  NumberOfTableDimensions=1  BreakpointsForDimension1=time_sl_taskmode  Table=algo_curPathPoint_LLA_0  InternalRulePriority=Speed  RndMeth=Simplest  InputSameDT=on
  algo_curPathPoint_LLA_1 : Lookup_n-D  NumberOfTableDimensions=1  BreakpointsForDimension1=time_sl_taskmode  Table=algo_curPathPoint_LLA_1  InternalRulePriority=Speed  RndMeth=Simplest  InputSameDT=on
  algo_curPosNED_0 : Lookup_n-D  NumberOfTableDimensions=1  BreakpointsForDimension1=time_sl_task_flight  Table=algo_curPosNED_0  InternalRulePriority=Speed  RndMeth=Simplest  InputSameDT=on
  algo_curPosNED_1 : Lookup_n-D  NumberOfTableDimensions=1  BreakpointsForDimension1=time_sl_task_flight  Table=algo_curPosNED_1  InternalRulePriority=Speed  RndMeth=Simplest  InputSameDT=on
  algo_curVelNED_0 : Lookup_n-D  NumberOfTableDimensions=1  BreakpointsForDimension1=time_sl_task_flight  Table=algo_curVelNED_0  InternalRulePriority=Speed  RndMeth=Simplest  InputSameDT=on
  algo_curVelNED_1 : Lookup_n-D  NumberOfTableDimensions=1  BreakpointsForDimension1=time_sl_task_flight  Table=algo_curVelNED_1  InternalRulePriority=Speed  RndMeth=Simplest  InputSameDT=on
  algo_curr_alt : Lookup_n-D  NumberOfTableDimensions=1  BreakpointsForDimension1=time_algo  Table=algo_curr_alt  InternalRulePriority=Speed  RndMeth=Simplest  InputSameDT=on
  algo_curr_pos_0 : Lookup_n-D  NumberOfTableDimensions=1  BreakpointsForDimension1=time_algo  Table=algo_curr_pos_0  InternalRulePriority=Speed  RndMeth=Simplest  InputSameDT=on
  algo_curr_pos_1 : Lookup_n-D  NumberOfTableDimensions=1  BreakpointsForDimension1=time_algo  Table=algo_curr_pos_1  InternalRulePriority=Speed  RndMeth=Simplest  InputSameDT=on
  algo_curr_vel_0 : Lookup_n-D  NumberOfTableDimensions=1  BreakpointsForDimension1=time_algo  Table=algo_curr_vel_0  InternalRulePriority=Speed  RndMeth=Simplest  InputSameDT=on
  algo_curr_vel_1 : Lookup_n-D  NumberOfTableDimensions=1  BreakpointsForDimension1=time_algo  Table=algo_curr_vel_1  InternalRulePriority=Speed  RndMeth=Simplest  InputSameDT=on
  algo_curr_vel_2 : Lookup_n-D  NumberOfTableDimensions=1  BreakpointsForDimension1=time_algo  Table=algo_curr_vel_2  InternalRulePriority=Speed  RndMeth=Simplest  InputSameDT=on
  algo_current_loc_0 : Lookup_n-D  NumberOfTableDimensions=1  BreakpointsForDimension1=time_algo  Table=algo_current_loc_0  InternalRulePriority=Speed  RndMeth=Simplest  InputSameDT=on
  algo_current_loc_1 : Lookup_n-D  NumberOfTableDimensions=1  BreakpointsForDimension1=time_algo  Table=algo_current_loc_1  InternalRulePriority=Speed  RndMeth=Simplest  InputSameDT=on
  algo_dbg_param : DataStoreMemory  DataStoreName=algo_dbg_param  ReadBeforeWriteMsg=warning  WriteAfterWriteMsg=warning  WriteAfterReadMsg=warning  InitialValue=algo_dbg_param  VectorParams1D=off  ShowAdditionalParam=off  OutDataTypeStr=Bus: BUS_CTRL_dbg_param
  algo_flightControlMode : Lookup_n-D  NumberOfTableDimensions=1  BreakpointsForDimension1=time_sl_taskmode  Table=algo_flightControlMode  InterpMethod=Flat  InternalRulePriority=Speed  OutDataTypeStr=uint8  RndMeth=Simplest  InputSameDT=on
  algo_flightTaskMode : Lookup_n-D  NumberOfTableDimensions=1  BreakpointsForDimension1=time_algo  Table=algo_flightTaskMode  InterpMethod=Flat  InternalRulePriority=Speed  OutDataTypeStr=uint8  RndMeth=Simplest  InputSameDT=on
  algo_heightCmd : Lookup_n-D  NumberOfTableDimensions=1  BreakpointsForDimension1=time_sl_taskmode  Table=algo_heightCmd_sl  InternalRulePriority=Speed  RndMeth=Simplest  InputSameDT=on
  algo_hgt_dem : Lookup_n-D  NumberOfTableDimensions=1  BreakpointsForDimension1=time_algo  Table=algo_hgt_dem  InternalRulePriority=Speed  RndMeth=Simplest  InputSameDT=on
  algo_k_aileron : Lookup_n-D  NumberOfTableDimensions=1  BreakpointsForDimension1=time_algo  Table=algo_k_aileron  InternalRulePriority=Speed  RndMeth=Simplest  InputSameDT=on
  algo_k_elevator : Lookup_n-D  NumberOfTableDimensions=1  BreakpointsForDimension1=time_algo  Table=algo_k_elevator  InternalRulePriority=Speed  RndMeth=Simplest  InputSameDT=on
  algo_k_rudder : Lookup_n-D  NumberOfTableDimensions=1  BreakpointsForDimension1=time_algo  Table=algo_k_rudder  InternalRulePriority=Speed  RndMeth=Simplest  InputSameDT=on
  algo_k_throttle : Lookup_n-D  NumberOfTableDimensions=1  BreakpointsForDimension1=time_algo  Table=algo_k_throttle  InternalRulePriority=Speed  RndMeth=Simplest  InputSameDT=on
  algo_latAccDem : Lookup_n-D  NumberOfTableDimensions=1  BreakpointsForDimension1=time_algo  Table=algo_latAccDem  InternalRulePriority=Speed  RndMeth=Simplest  InputSameDT=on
  algo_limit_pos_up : Lookup_n-D  NumberOfTableDimensions=1  BreakpointsForDimension1=time_algo  Table=algo_limit_pos_up  InternalRulePriority=Speed  RndMeth=Simplest  InputSameDT=on
  algo_maxClimbSpeed : Lookup_n-D  NumberOfTableDimensions=1  BreakpointsForDimension1=time_algo  Table=algo_maxClimbSpeed  InterpMethod=Flat  InternalRulePriority=Speed  OutDataTypeStr=double  RndMeth=Simplest  InputSameDT=on
  algo_mode : Lookup_n-D  NumberOfTableDimensions=1  BreakpointsForDimension1=time_algo  Table=algo_mode  IntermediateResultsDataTypeStr=uint8  InterpMethod=Nearest  ExtrapMethod=Clip  InternalRulePriority=Speed  OutDataTypeStr=uint8  RndMeth=Simplest  InputSameDT=on
  algo_nav_pitch_cd : Lookup_n-D  NumberOfTableDimensions=1  BreakpointsForDimension1=time_algo  Table=algo_nav_pitch_cd  InternalRulePriority=Speed  RndMeth=Simplest  InputSameDT=on
  algo_nav_roll : Lookup_n-D  NumberOfTableDimensions=1  BreakpointsForDimension1=time_algo  Table=algo_nav_roll  InternalRulePriority=Speed  RndMeth=Simplest  InputSameDT=on
  algo_pitch_dem : Lookup_n-D  NumberOfTableDimensions=1  BreakpointsForDimension1=time_algo  Table=algo_pitch_dem  InternalRulePriority=Speed  RndMeth=Simplest  InputSameDT=on
  algo_pitch_in : Lookup_n-D  NumberOfTableDimensions=1  BreakpointsForDimension1=time_algo  Table=algo_pitch_in  InternalRulePriority=Speed  RndMeth=Simplest  InputSameDT=on
  algo_pitch_target_pilot : Lookup_n-D  NumberOfTableDimensions=1  BreakpointsForDimension1=time_algo  Table=algo_pitch_target_pilot  InternalRulePriority=Speed  RndMeth=Simplest  InputSameDT=on
  algo_plane_mode : Lookup_n-D  NumberOfTableDimensions=1  BreakpointsForDimension1=time_sl_taskmode  Table=algo_plane_mode  InterpMethod=Flat  InternalRulePriority=Speed  OutDataTypeStr=uint8  RndMeth=Simplest  InputSameDT=on
  algo_pos_target_0 : Lookup_n-D  NumberOfTableDimensions=1  BreakpointsForDimension1=time_algo  Table=algo_pos_target_0  InternalRulePriority=Speed  RndMeth=Simplest  InputSameDT=on
  algo_pos_target_1 : Lookup_n-D  NumberOfTableDimensions=1  BreakpointsForDimension1=time_algo  Table=algo_pos_target_1  InternalRulePriority=Speed  RndMeth=Simplest  InputSameDT=on
  algo_pos_target_2 : Lookup_n-D  NumberOfTableDimensions=1  BreakpointsForDimension1=time_algo  Table=algo_pos_target_2  InternalRulePriority=Speed  RndMeth=Simplest  InputSameDT=on
  algo_prePathPoint_LLA_0 : Lookup_n-D  NumberOfTableDimensions=1  BreakpointsForDimension1=time_sl_taskmode  Table=algo_prePathPoint_LLA_0  InternalRulePriority=Speed  RndMeth=Simplest  InputSameDT=on
  algo_prePathPoint_LLA_1 : Lookup_n-D  NumberOfTableDimensions=1  BreakpointsForDimension1=time_sl_taskmode  Table=algo_prePathPoint_LLA_1  InternalRulePriority=Speed  RndMeth=Simplest  InputSameDT=on
  algo_pwm_out_1 : Lookup_n-D  NumberOfTableDimensions=1  BreakpointsForDimension1=time_algo  Table=algo_pwm_out_1  InternalRulePriority=Speed  RndMeth=Simplest  InputSameDT=on
  algo_pwm_out_2 : Lookup_n-D  NumberOfTableDimensions=1  BreakpointsForDimension1=time_algo  Table=algo_pwm_out_2  InternalRulePriority=Speed  RndMeth=Simplest  InputSameDT=on
  algo_pwm_out_3 : Lookup_n-D  NumberOfTableDimensions=1  BreakpointsForDimension1=time_algo  Table=algo_pwm_out_3  InternalRulePriority=Speed  RndMeth=Simplest  InputSameDT=on
  algo_pwm_out_4 : Lookup_n-D  NumberOfTableDimensions=1  BreakpointsForDimension1=time_algo  Table=algo_pwm_out_4  InternalRulePriority=Speed  RndMeth=Simplest  InputSameDT=on
  algo_rate_target_ang_vel_0 : Lookup_n-D  NumberOfTableDimensions=1  BreakpointsForDimension1=time_algo  Table=algo_rate_target_ang_vel_0  InternalRulePriority=Speed  RndMeth=Simplest  InputSameDT=on
  algo_rate_target_ang_vel_1 : Lookup_n-D  NumberOfTableDimensions=1  BreakpointsForDimension1=time_algo  Table=algo_rate_target_ang_vel_1  InternalRulePriority=Speed  RndMeth=Simplest  InputSameDT=on
  algo_rate_target_ang_vel_2 : Lookup_n-D  NumberOfTableDimensions=1  BreakpointsForDimension1=time_algo  Table=algo_rate_target_ang_vel_2  InternalRulePriority=Speed  RndMeth=Simplest  InputSameDT=on
  algo_remote_ct_st : DataStoreMemory  DataStoreName=algo_remote_ct_st  ReadBeforeWriteMsg=warning  WriteAfterWriteMsg=warning  WriteAfterReadMsg=warning  InitialValue=algo_remote_ct_st  VectorParams1D=off  ShowAdditionalParam=off  OutDataTypeStr=Bus:BUS_CTRL_remote_ct_st
  algo_remote_ct_st_pitch : Lookup_n-D  NumberOfTableDimensions=1  BreakpointsForDimension1=time_algo  Table=algo_remote_ct_st_pitch  InternalRulePriority=Speed  RndMeth=Simplest  InputSameDT=on
  algo_remote_ct_st_roll : Lookup_n-D  NumberOfTableDimensions=1  BreakpointsForDimension1=time_algo  Table=algo_remote_ct_st_roll  InternalRulePriority=Speed  RndMeth=Simplest  InputSameDT=on
  algo_remote_ct_st_throttle : Lookup_n-D  NumberOfTableDimensions=1  BreakpointsForDimension1=time_algo  Table=algo_throttle_in  InternalRulePriority=Speed  RndMeth=Simplest  InputSameDT=on
  algo_remote_ct_st_yaw : Lookup_n-D  NumberOfTableDimensions=1  BreakpointsForDimension1=time_algo  Table=algo_remote_ct_st_yaw  InternalRulePriority=Speed  RndMeth=Simplest  InputSameDT=on
  algo_rollCmd : Lookup_n-D  NumberOfTableDimensions=1  BreakpointsForDimension1=time_sl_taskmode  Table=algo_rollCmd  IntermediateResultsDataTypeStr=uint8  InterpMethod=Nearest  ExtrapMethod=Clip  InternalRulePriority=Speed  RndMeth=Simplest  InputSameDT=on
  algo_roll_in : Lookup_n-D  NumberOfTableDimensions=1  BreakpointsForDimension1=time_algo  Table=algo_roll_in  InternalRulePriority=Speed  RndMeth=Simplest  InputSameDT=on
  algo_roll_target_pilot : Lookup_n-D  NumberOfTableDimensions=1  BreakpointsForDimension1=time_algo  Table=algo_roll_target_pilot  InternalRulePriority=Speed  RndMeth=Simplest  InputSameDT=on
  algo_tail_tilt : Lookup_n-D  NumberOfTableDimensions=1  BreakpointsForDimension1=time_algo  Table=algo_tail_tilt  InternalRulePriority=Speed  RndMeth=Simplest  InputSameDT=on
  algo_throttle_dem : Lookup_n-D  NumberOfTableDimensions=1  BreakpointsForDimension1=time_algo  Table=algo_throttle_dem  InternalRulePriority=Speed  RndMeth=Simplest  InputSameDT=on
  algo_throttle_filter : Lookup_n-D  NumberOfTableDimensions=1  BreakpointsForDimension1=time_algo  Table=algo_throttle_filter  InternalRulePriority=Speed  RndMeth=Simplest  InputSameDT=on
  algo_throttle_in : Lookup_n-D  NumberOfTableDimensions=1  BreakpointsForDimension1=time_algo  Table=algo_throttle_in  InternalRulePriority=Speed  RndMeth=Simplest  InputSameDT=on
  algo_throttle_lower : Lookup_n-D  NumberOfTableDimensions=1  BreakpointsForDimension1=time_algo  Table=algo_throttle_lower  InternalRulePriority=Speed  RndMeth=Simplest  InputSameDT=on
  algo_throttle_upper : Lookup_n-D  NumberOfTableDimensions=1  BreakpointsForDimension1=time_algo  Table=algo_throttle_upper  InternalRulePriority=Speed  RndMeth=Simplest  InputSameDT=on
  algo_turnCenterLL_0 : Lookup_n-D  NumberOfTableDimensions=1  BreakpointsForDimension1=time_sl_taskmode  Table=algo_turnCenterLL_0  InternalRulePriority=Speed  RndMeth=Simplest  InputSameDT=on
  algo_turnCenterLL_1 : Lookup_n-D  NumberOfTableDimensions=1  BreakpointsForDimension1=time_sl_taskmode  Table=algo_turnCenterLL_1  InternalRulePriority=Speed  RndMeth=Simplest  InputSameDT=on
  algo_vel_desired_2 : Lookup_n-D  NumberOfTableDimensions=1  BreakpointsForDimension1=time_algo  Table=algo_vel_desired_2  InternalRulePriority=Speed  RndMeth=Simplest  InputSameDT=on
  algo_vel_target_0 : Lookup_n-D  NumberOfTableDimensions=1  BreakpointsForDimension1=time_algo  Table=algo_vel_target_0  InternalRulePriority=Speed  RndMeth=Simplest  InputSameDT=on
  algo_vel_target_1 : Lookup_n-D  NumberOfTableDimensions=1  BreakpointsForDimension1=time_algo  Table=algo_vel_target_1  InternalRulePriority=Speed  RndMeth=Simplest  InputSameDT=on
  algo_vel_target_2 : Lookup_n-D  NumberOfTableDimensions=1  BreakpointsForDimension1=time_algo  Table=algo_vel_target_2  InternalRulePriority=Speed  RndMeth=Simplest  InputSameDT=on
  algo_weathervane_last_output : Lookup_n-D  NumberOfTableDimensions=1  BreakpointsForDimension1=time_algo  Table=algo_weathervane_last_output  InternalRulePriority=Speed  RndMeth=Simplest  InputSameDT=on
  algo_yaw_in : Lookup_n-D  NumberOfTableDimensions=1  BreakpointsForDimension1=time_algo  Table=algo_yaw_in  InternalRulePriority=Speed  RndMeth=Simplest  InputSameDT=on
  algo_z_accel_meas : Lookup_n-D  NumberOfTableDimensions=1  BreakpointsForDimension1=time_algo  Table=algo_z_accel_meas  InternalRulePriority=Speed  RndMeth=Simplest  InputSameDT=on
  ax_f : Lookup_n-D  NumberOfTableDimensions=1  BreakpointsForDimension1=time_algo  Table=ax_f  InternalRulePriority=Speed  RndMeth=Simplest  InputSameDT=on
  ay_f : Lookup_n-D  NumberOfTableDimensions=1  BreakpointsForDimension1=time_algo  Table=ay_f  InternalRulePriority=Speed  RndMeth=Simplest  InputSameDT=on
  az_f : Lookup_n-D  NumberOfTableDimensions=1  BreakpointsForDimension1=time_algo  Table=az_f  InternalRulePriority=Speed  RndMeth=Simplest  InputSameDT=on
  b2e : Product  Multiplication=Matrix(*)  InputSameDT=on  SaturateOnIntegerOverflow=on  OutDataTypeStr=Inherit: Same as first input
  b2e2 : Product  Multiplication=Matrix(*)  InputSameDT=on  SaturateOnIntegerOverflow=on  OutDataTypeStr=Inherit: Same as first input
  dt1 : DataStoreMemory  DataStoreName=dt  ReadBeforeWriteMsg=warning  WriteAfterWriteMsg=warning  WriteAfterReadMsg=warning  InitialValue=dt  ShowAdditionalParam=off  OutDataTypeStr=double
  e2b : Product  Multiplication=Matrix(*)  InputSameDT=on  SaturateOnIntegerOverflow=on  OutDataTypeStr=Inherit: Same as first input
  gn2 : Constant  Value=[0;0;GRAVITY_MSS]
  gx_f2 : Lookup_n-D  NumberOfTableDimensions=1  BreakpointsForDimension1=time_algo  Table=gx_f  InternalRulePriority=Speed  RndMeth=Simplest  InputSameDT=on
  gy_f2 : Lookup_n-D  NumberOfTableDimensions=1  BreakpointsForDimension1=time_algo  Table=gy_f  InternalRulePriority=Speed  RndMeth=Simplest  InputSameDT=on
  gz_f2 : Lookup_n-D  NumberOfTableDimensions=1  BreakpointsForDimension1=time_algo  Table=gz_f  InternalRulePriority=Speed  RndMeth=Simplest  InputSameDT=on
  input_euler_angle_roll_pitch_euler_rate_yaw : MATLAB Function  TreatAsAtomicUnit=on
  pitch_t : Lookup_n-D  NumberOfTableDimensions=1  BreakpointsForDimension1=time_algo  Table=algo_pitch  InternalRulePriority=Speed  RndMeth=Simplest  InputSameDT=on
  plane_mode : DataStoreMemory  DataStoreName=plane_mode  ReadBeforeWriteMsg=warning  WriteAfterWriteMsg=warning  WriteAfterReadMsg=warning  InitialValue=plane_mode  VectorParams1D=off  ShowAdditionalParam=off  OutDataTypeStr=Enum: ENUM_plane_mode
  roll_t : Lookup_n-D  NumberOfTableDimensions=1  BreakpointsForDimension1=time_algo  Table=algo_roll  InternalRulePriority=Speed  RndMeth=Simplest  InputSameDT=on
  systime : DataStoreMemory  DataStoreName=systime  ReadBeforeWriteMsg=warning  WriteAfterWriteMsg=warning  WriteAfterReadMsg=warning  InitialValue=systime  ShowAdditionalParam=off  OutDataTypeStr=double
  yaw_t : Lookup_n-D  NumberOfTableDimensions=1  BreakpointsForDimension1=time_algo  Table=algo_yaw  InternalRulePriority=Speed  RndMeth=Simplest  InputSameDT=on
  Out1 : Outport  OutDataTypeStr=Bus: BUS_CTRL_SRV_Channel
  wires:
  Data Store Read/1 -> Out1/1
  NAVI2CONTROL/1 -> Bus Selector1/1
  Bus Selector1/3 -> Data Type Conversion2/1  "<yawd>"
  Bus Selector/2 -> Data Store Write2/4  "<curLLA>"
  Bus Selector3/2 -> Data Type Conversion4/1  "<EAS2TAS_Algo>"
  Bus Selector2/2 -> Data Type Conversion6/1  "<gyro_y>"
  Bus Selector2/4 -> Data Type Conversion8/1  "<accel_x>"
  PathModeOut/1 -> Data Store Write2/9  "PathModeOut"
  Bus Selector2/6 -> Data Type Conversion10/1  "<accel_z>"
  Bus Selector2/1 -> Data Type Conversion5/1  "<gyro_x>"
  TASK_COMMON_OutParam/1 -> Bus Selector/1
  Bus Selector2/3 -> Data Type Conversion7/1  "<gyro_z>"
  CTRL_wp/1 -> Data Store Write2/10  "wp_in"
  Bus Selector/1 -> Data Store Write2/3  "<curVelNED>"
  EAS_Algo/1 -> Bus Selector3/1  "EAS_Algo"
  Bus Selector1/2 -> Data Type Conversion1/1  "<rolld>"
  Data Type Conversion4/1 -> Data Store Write2/2  "EAS2TAS_Algo"
  Data Type Conversion/1 -> Data Store Write2/5  "pitchd"
  Bus Selector1/4 -> Data Type Conversion11/1  "<alt>"
  Data Type Conversion2/1 -> Data Store Write2/7  "yawd"
  Data Type Conversion1/1 -> Data Store Write2/6  "rolld"
  Bus Selector1/1 -> Data Type Conversion/1  "<pitchd>"
  Data Type Conversion3/1 -> Data Store Write2/1  "EAS_Algo"
  Bus Selector3/1 -> Data Type Conversion3/1  "<airspeed_indicate>"
  Data Type Conversion5/1 -> ?  "gyro_x"
  Data Type Conversion6/1 -> ?  "gyro_y"
  IMU/1 -> Bus Selector2/1
  Data Type Conversion8/1 -> ?  "accel_x"
  Data Type Conversion11/1 -> Data Store Write2/8  "NAV_alt"
  Bus Selector2/5 -> Data Type Conversion9/1  "<accel_y>"
  Data Type Conversion7/1 -> ?  "gyro_z"
  Data Type Conversion9/1 -> ?  "accel_y"
  Data Type Conversion10/1 -> ?  "accel_z"
  Data Store Read21/6 -> Scope35/1
  "Incidence, Sideslip & Airspeed3"/2 -> Gain37/1  "Beta"
  Data Store Read21/10 -> Scope39/1
  Data Store Read21/8 -> Scope37/1
  Data Store Read21/4 -> Scope33/1
  Data Store Read21/1 -> Scope30/1
  Data Store Read18/1 -> Display5/1
  Data Store Read60/1 -> Display1/1
  Data Store Read21/7 -> Scope36/1
  "Incidence, Sideslip & Airspeed3"/3 -> Scope71/1
  Data Store Read21/2 -> Scope31/1
  Data Store Read21/9 -> Scope38/1
  Data Store Read21/3 -> Scope32/1
  "Incidence, Sideslip & Airspeed3"/1 -> Gain49/1  "alpha"
  [Vb] -> "Incidence, Sideslip & Airspeed3"/1
  Data Store Read21/5 -> Scope34/1
  Gain37/1 -> Scope68/1
  Gain49/1 -> Scope67/1
  Data Store Read14/2 -> Scope107/1
  Data Store Read14/1 -> Scope120/1
  Data Store Read14/4 -> Scope109/1
  Data Store Read14/3 -> Scope108/1
  Data Store Read14/6 -> Scope133/1
  Data Store Read14/5 -> Scope125/1
  Data Store Read14/8 -> Scope15/1
  Data Store Read14/7 -> Scope136/1
  Data Store Read56/1 -> Display6/1
  Constant1/1 -> Data Store Write4/1
  Data Store Read57/1 -> Gain31/1
  Data Store Read57/2 -> Gain30/1
  Data Store Read57/3 -> Gain32/1
  Gain31/1 -> Scope22/1
  Gain30/1 -> Scope116/1
  Gain32/1 -> Scope119/1
  Gain35/1 -> Scope130/1
  Gain33/1 -> Scope129/1
  Gain34/1 -> Scope131/1
  Data Store Read62/3 -> Gain35/1
  Data Store Read62/2 -> Gain33/1
  Data Store Read62/1 -> Gain34/1
  Data Store Read63/1 -> Gain43/1
  Data Store Read63/2 -> Gain36/1
  Data Store Read63/3 -> Gain48/1
  Gain43/1 -> Scope146/1
  Gain36/1 -> Scope141/1
  Gain48/1 -> Scope144/1
  Data Store Read64/1 -> Scope152/1
  Constant9/1 -> Data Store Write12/1
  Data Store Read1/9 -> Gain61/1
  Data Store Read1/6 -> Scope92/1
  Data Store Read1/4 -> Scope178/1
  Data Store Read1/12 -> Scope17/1
  Data Store Read1/14 -> Scope23/1
  Data Store Read1/5 -> Scope86/1
  Data Store Read1/7 -> Gain59/1
  Data Store Read1/16 -> Scope27/1
  Data Store Read1/11 -> Scope24/1
  Data Store Read1/13 -> Scope19/1
  Data Store Read1/15 -> Scope26/1
  Data Store Read1/17 -> Scope66/1
  Data Store Read1/2 -> Gain63/1
  Data Store Read1/3 -> Gain64/1
  Data Store Read1/1 -> Gain62/1
  Gain64/1 -> Scope177/1
  Gain62/1 -> Scope65/1
  Gain63/1 -> Scope175/1
  Data Store Read1/8 -> Gain60/1
  Data Store Read1/10 -> Scope132/1
  Gain60/1 -> Scope115/1
  Gain59/1 -> Scope93/1
  Gain61/1 -> Scope123/1
  Constant10/1 -> Data Store Write14/1
  Data Store Read68/1 -> Demux3/1
  Data Store Read71/1 -> Demux4/1
  Data Store Read74/1 -> Demux9/1
  Data Store Read108/1 -> Demux12/1
  Data Store Read107/1 -> Demux13/1
  Demux3/1 -> Scope2/1
  Demux3/2 -> Scope2/2
  Demux3/3 -> Scope2/3
  Demux4/1 -> Scope159/1
  Demux4/2 -> Scope159/2
  Demux4/3 -> Scope159/3
  Demux9/1 -> Scope161/1
  Demux9/2 -> Scope161/2
  Demux9/3 -> Scope161/3
  Demux12/1 -> Scope164/1
  Demux12/2 -> Scope164/2
  Demux12/3 -> Scope164/3
  Demux13/1 -> Scope165/1
  Demux13/2 -> Scope165/2
  Demux13/3 -> Scope165/3
  Data Store Read114/1 -> Scope169/1
  Data Store Read116/1 -> Scope169/2
  Demux21/1 -> Scope167/1
  Demux22/3 -> Scope168/2
  Demux22/1 -> Scope167/2
  Demux22/2 -> Scope166/2
  Demux21/2 -> Scope166/1
  Data Store Read112/1 -> Demux21/1
  Data Store Read109/1 -> Demux22/1
  Demux21/3 -> Scope168/1
  Data Store Read117/1 -> Scope171/3
  Data Store Read118/1 -> Scope171/1
  Data Store Read119/1 -> Scope172/1
  Data Store Read120/1 -> Scope172/2
  Data Store Read135/1 -> Scope174/2
  Data Store Read8/1 -> Divide4/1
  Data Store Read8/2 -> Divide4/2
  Data Store Read8/3 -> Divide5/1
  Data Store Read8/4 -> Divide5/2
  Divide5/1 -> Scope173/2, Add9/2  "D"
  Divide4/1 -> Scope173/1, Add9/1  "P"
  Data Store Read132/1 -> Add10/2, Scope249/2
  Data Store Read137/1 -> Scope249/3, Add10/3
  Add10/1 -> Scope174/1
  Gain65/1 -> Scope249/1, Add10/1
  Data Store Read125/1 -> Scope179/2
  Data Store Read124/1 -> Scope179/1
  Data Store Read123/1 -> Scope78/1
  Data Store Read90/1 -> Scope78/2
  Data Store Read140/1 -> Scope183/2
  Data Store Read10/1 -> Scope183/1
  Data Store Read11/1 -> Scope8/1
  Data Store Read139/1 -> Scope8/2
  Add3/1 -> Gain70/1
  b2e/1 -> Add3/1
  Selector2/1 -> Rotation Angles to Direction Cosine Matrix1/1
  Transpose3/1 -> b2e/1
  gn2/1 -> Add3/2
  Mux7/1 -> Selector2/1
  Rotation Angles to Direction Cosine Matrix1/1 -> e2b/1, b2e2/1, Transpose3/1
  Data Store Read174/3 -> Mux7/3
  Data Store Read174/2 -> Mux7/2
  Data Store Read174/1 -> Mux7/1
  Data Store Read171/1 -> Mux3/1
  Data Store Read171/2 -> Mux3/2
  Data Store Read171/3 -> Mux3/3
  Mux3/1 -> b2e/2
  Demux24/1 -> Scope186/2
  Demux24/2 -> Scope187/2
  Gain70/1 -> b2e2/2, Scope184/1
  Data Store Read172/2 -> Mux10/2, MATLAB Function17/2(y_cmss)
  Data Store Read172/3 -> Mux10/3
  Mux10/1 -> e2b/2
  e2b/1 -> Demux25/1
  b2e2/1 -> Demux24/1
  Data Store Read76/1 -> Gain18/1
  Gain18/1 -> Tan/1
  Tan/1 -> Gain23/1
  Gain23/1 -> Gain24/1
  Gain24/1 -> Scope206/1
  Divide1/1 -> Scope207/1
  Gain50/1 -> Divide1/2
  Gain20/1 -> Tan2/1
  Tan2/1 -> Divide1/1
  Data Store Read92/1 -> Gain20/1
  Data Store Read91/1 -> Gain25/1
  Gain27/1 -> Gain50/1
  Gain25/1 -> Tan1/1
  Tan1/1 -> Gain27/1
  Data Store Read172/1 -> Mux10/1, MATLAB Function17/1(x_cmss)
  MATLAB Function17/1(forward) -> Scope186/1, Scope206/2
  MATLAB Function17/2(right) -> Scope187/1, Scope207/2
  Data Store Read22/1 -> Gain9/1
  Data Store Read23/1 -> Gain11/1
  Data Store Read22/2 -> Gain10/1
  Data Store Read23/2 -> Gain12/1
  Gain9/1 -> Scope76/1
  Gain10/1 -> Scope77/1
  Gain11/1 -> Scope76/2
  Gain12/1 -> Scope77/2
  Data Store Read24/1 -> Scope79/1
  Data Store Read24/2 -> Scope82/1
  Data Store Read24/3 -> Scope89/1
  Data Store Read24/4 -> Scope90/1
  Data Store Read24/5 -> Scope91/1
  Data Store Read24/6 -> Scope94/1
  Data Store Read24/7 -> Scope101/1
  Data Store Read25/1 -> Display7/1
  Data Store Read26/3 -> Scope21/1
  Data Store Read26/1 -> Scope4/1
  Data Store Read26/2 -> Scope20/1
  Data Store Read19/2 -> Scope16/1
  Data Store Read19/4 -> Scope95/1
  Data Store Read19/1 -> Scope111/1
  Data Store Read19/3 -> Scope18/1
  Data Store Read19/5 -> Scope112/1
  Data Store Read19/6 -> Scope104/1
  Data Store Read30/1 -> Divide12/1
  Data Store Read30/3 -> Divide13/1
  Divide12/1 -> Scope53/1, Add13/1  "P"
  Divide13/1 -> Add13/2, Scope53/2  "D"
  Data Store Read30/2 -> Divide12/2
  Add13/1 -> Scope149/1
  Data Store Read30/5 -> Scope53/3, Add13/3  "I"
  Data Store Read30/4 -> Divide13/2
  Data Store Read27/1 -> Scope149/2
  Data Store Read28/1 -> Scope153/2
  Data Store Read29/4 -> Divide15/2
  Data Store Read29/5 -> Add12/3, Scope156/3  "I"
  Add12/1 -> Scope153/1
  Data Store Read29/2 -> Divide14/2
  Divide15/1 -> Scope156/2, Add12/2  "D"
  Divide14/1 -> Add12/1, Scope156/1  "P"
  Data Store Read29/3 -> Divide15/1
  Data Store Read29/1 -> Divide14/1
  Data Store Read118/2 -> Scope171/2
  Gain13/1 -> Scope185/1
  Gain86/1 -> Scope196/1, Scope198/1
  Data Store Read9/1 -> Divide10/1
  Gain82/1 -> Scope192/1, Scope199/2
  Data Store Read9/6 -> Scope10/3, Add11/3  "I"
  Data Store Read15/1 -> Scope52/2
  Divide8/1 -> Add6/1, Scope7/1  "P"
  Data Store Read6/1 -> Scope9/2
  Data Store Read3/3 -> Divide7/1
  Data Store Read31/1 -> Gain13/1
  Data Store Read9/2 -> Divide10/2
  Data Store Read5/1 -> Divide8/1
  Gain66/1 -> Scope202/1, Scope180/1
  Data Store Read3/6 -> Scope5/3, Add4/3  "I"
  Gain67/1 -> Scope201/1, Scope182/1
  Data Store Read4/1 -> Scope6/2
  Data Store Read142/1 -> Gain83/1
  Add11/1 -> Scope52/1
  Data Store Read5/6 -> Add6/3, Scope7/3  "I"
  Gain68/1 -> Scope203/1, Scope181/1
  Data Store Read9/5 -> Scope275/1, Divide10/3, Divide11/3
  Add4/1 -> Scope6/1
  Divide11/1 -> Scope10/2, Add11/2  "D"
  Data Store Read3/4 -> Divide7/2
  Data Store Read5/3 -> Divide9/1
  Divide9/1 -> Add6/2, Scope7/2  "D"
  Gain75/1 -> Scope189/1, Scope202/2
  Data Store Read5/5 -> Divide9/3, Divide8/3, Scope273/1
  Data Store Read5/2 -> Divide8/2
  Data Store Read5/4 -> Divide9/2
  Divide10/1 -> Scope10/1, Add11/1  "P"
  Divide7/1 -> Scope5/2, Add4/2  "D"
  Data Store Read9/4 -> Divide11/2
  Divide6/1 -> Scope5/1, Add4/1  "P"
  Data Store Read3/2 -> Divide6/2
  Data Store Read141/1 -> Gain80/1
  Data Store Read141/3 -> Gain81/1
  Data Store Read138/1 -> Gain67/1
  Gain87/1 -> Scope199/1, Scope197/1
  Data Store Read166/1 -> Gain86/1
  Data Store Read167/1 -> Gain85/1
  Data Store Read3/1 -> Divide6/1
  Gain85/1 -> Scope200/1, Scope195/1
  Data Store Read9/3 -> Divide11/1
  Gain83/1 -> Scope194/1, Scope198/2
  Gain81/1 -> Scope203/2, Scope190/1
  Data Store Read142/3 -> Gain84/1
  Data Store Read142/2 -> Gain82/1
  Gain84/1 -> Scope200/2, Scope193/1
  Data Store Read141/2 -> Gain75/1
  Data Store Read166/2 -> Gain87/1
  Add6/1 -> Scope9/1
  Gain80/1 -> Scope201/2, Scope191/1
  Data Store Read138/3 -> Gain68/1
  Data Store Read138/2 -> Gain66/1
  Data Store Read3/5 -> Scope274/1, Divide6/3, Divide7/3
  Data Store Read75/1 -> Gain15/1
  Gain15/1 -> Scope208/2
  Data Store Read82/1 -> Gain16/1
  Gain16/1 -> Scope209/2
  Data Store Read70/1 -> Gain19/1
  Data Store Read49/1 -> Gain17/1
  Gain17/1 -> Scope208/1
  Gain19/1 -> Scope209/1
  Data Store Read97/1 -> Gain51/1
  Data Store Read97/2 -> Gain53/1
  Data Store Read97/3 -> Scope212/1
  Data Store Read97/4 -> Scope213/1
  Data Store Read97/5 -> Scope214/1
  Data Store Read97/6 -> Scope215/1
  Gain51/1 -> Scope210/1
  Gain53/1 -> Scope211/1
  Add/1 -> Scope216/1
  Data Store Read99/6 -> Scope216/2
  Data Store Read97/13 -> Scope223/1
  Data Store Read97/14 -> Scope224/1
  Data Store Read97/7 -> Scope217/1
  Data Store Read97/8 -> Scope218/1
  Data Store Read97/9 -> Scope219/1
  Data Store Read97/10 -> Scope220/1
  Data Store Read97/11 -> Scope221/1
  Data Store Read97/12 -> Scope222/1
  Data Store Read99/1 -> Scope237/1, Add/1  "P"
  Data Store Read99/2 -> Add/2, Scope237/2  "I"
  Data Store Read99/3 -> Scope237/3, Add/3  "D"
  Data Store Read99/4 -> Scope237/4, Add/4  "FF"
  Data Store Read99/5 -> Scope225/1
  Data Store Read100/5 -> Scope227/1
  Data Store Read100/4 -> Scope238/4, Add14/4  "FF"
  Data Store Read100/3 -> Scope238/3, Add14/3  "D"
  Data Store Read100/2 -> Scope238/2, Add14/2  "I"
  Data Store Read100/1 -> Scope238/1, Add14/1  "P"
  Data Store Read100/6 -> Scope226/2
  Add14/1 -> Scope226/1
  Data Store Read101/1 -> Scope229/1, Add15/1  "I"
  Data Store Read101/3 -> Scope228/2
  Data Store Read101/2 -> Scope229/2, Add15/2  "D"
  Data Store Read105/1 -> Scope231/1
  Data Store Read105/2 -> Scope232/1
  Data Store Read105/3 -> Scope233/1
  Data Store Read105/4 -> Scope234/1
  Data Store Read105/5 -> Scope235/1
  Data Store Read98/1 -> Scope236/1
  Add15/1 -> Scope228/1
  Data Store Read144/1 -> Gain21/1
  Gain21/1 -> Scope230/2
  Data Store Read47/1 -> Scope230/1
  Data Store Read146/1 -> Scope239/1
  Data Store Read145/1 -> Scope239/2
  Data Store Read147/1 -> Scope240/1
  [Xe] -> Scope241/1
  Data Store Read148/2 -> Gain22/1
  Data Store Read148/3 -> Gain55/1
  Data Store Read148/1 -> Gain54/1
  Gain54/1 -> Scope244/1
  Gain22/1 -> Scope242/1
  Gain55/1 -> Scope243/1
  Data Store Read149/1 -> Scope245/1
  Gain73/1 -> Scope247/1
  Gain71/1 -> Scope246/1
  Gain72/1 -> Scope248/1
  Data Store Read152/1 -> Gain72/1
  Data Store Read152/3 -> Gain73/1
  Data Store Read152/2 -> Gain71/1
  Data Store Read8/6 -> Scope173/3, Scope251/2, Add16/2  "I"
  Add9/1 -> Derivative/1, Scope252/1, Divide16/1
  Divide16/1 -> Derivative3/1, Add16/1, Scope252/2, Scope251/1  "PD"
  Add16/1 -> Gain65/1
  Data Store Read8/5 -> Scope250/2, Divide16/2
  Derivative/1 -> Mux2/1
  Derivative3/1 -> Mux2/2
  Mux2/1 -> Scope250/1
  Data Store Read154/1 -> Scope254/1
  Data Store Read154/2 -> Scope253/1
  Data Store Read154/3 -> Scope255/1
  Data Store Read154/5 -> Scope256/1
  Data Store Read154/4 -> Scope257/1
  Data Store Read154/6 -> Scope258/1
  Data Store Read154/8 -> Scope259/1
  Data Store Read154/10 -> Scope263/1
  Data Store Read154/12 -> Scope264/1
  Data Store Read154/14 -> Scope265/1
  Data Store Read154/16 -> Scope269/1
  Data Store Read154/18 -> Scope270/1
  Data Store Read154/20 -> Scope271/1
  Data Store Read154/7 -> Scope260/1
  Data Store Read154/9 -> Scope261/1
  Data Store Read154/11 -> Scope262/1
  Data Store Read154/13 -> Scope266/1
  Data Store Read154/15 -> Scope267/1
  Data Store Read154/17 -> Scope268/1
  Data Store Read154/19 -> Scope272/1
  Constant27/1 -> Data Type Conversion14/1
  Data Type Conversion14/1 -> Data Store Write35/1
  Data Store Read2/1 -> Scope1/1
  Data Store Read7/1 -> Scope3/1
  Constant19/1 -> Data Store Write1/2
  Constant21/1 -> Data Store Write1/4
  Constant23/1 -> Data Store Write1/6
  Constant25/1 -> Data Store Write1/8
  Constant18/1 -> Data Store Write1/1
  Constant20/1 -> Data Store Write1/3
  Constant22/1 -> Data Store Write1/5
  Constant24/1 -> Data Store Write1/7
  Constant26/1 -> Data Store Write1/9
  Constant28/1 -> Data Store Write1/10
  Constant39/1 -> Data Store Write3/10
  Constant38/1 -> Data Store Write3/9
  Constant36/1 -> Data Store Write3/7
  Constant34/1 -> Data Store Write3/5
  Constant32/1 -> Data Store Write3/3
  Constant29/1 -> Data Store Write3/1
  Constant37/1 -> Data Store Write3/8
  Constant35/1 -> Data Store Write3/6
  Constant33/1 -> Data Store Write3/4
  Constant31/1 -> Data Store Write3/2
  Constant41/1 -> Data Store Write16/2
  Constant43/1 -> Data Store Write16/4
  Constant45/1 -> Data Store Write16/6
  Constant47/1 -> Data Store Write16/8
  Constant40/1 -> Data Store Write16/1
  Constant42/1 -> Data Store Write16/3
  Constant44/1 -> Data Store Write16/5
  Constant46/1 -> Data Store Write16/7
  Constant48/1 -> Data Store Write16/9
  Constant49/1 -> Data Store Write16/10
  algo_plane_mode/1 -> Data Type Conversion16/1
  algo_rollCmd/1 -> Data Store Write32/1
  algo_turnCenterLL_0/1 -> Data Store Write23/1
  algo_flightControlMode/1 -> Data Type Conversion17/1
  Data Type Conversion17/1 -> Data Store Write39/1, Scope143/1
  Data Type Conversion16/1 -> Scope29/1, Data Store Write38/1
  algo_flightTaskMode/1 -> Scope100/1, Data Type Conversion15/1
  ? -> ?
  Data Type Conversion15/1 -> Data Store Write21/1, Scope97/1
  algo_curPathPoint_LLA_1/1 -> Data Store Write31/1
  algo_curPathPoint_LLA_0/1 -> Data Store Write30/1
  algo_heightCmd/1 -> Data Store Write20/1
  algo_turnCenterLL_1/1 -> Data Store Write24/1
  algo_prePathPoint_LLA_1/1 -> Data Store Write26/1
  algo_remote_ct_st_roll/1 -> Data Store Write63/1
  ? -> ?
  algo_remote_ct_st_pitch/1 -> Data Store Write47/1
  algo_remote_ct_st_throttle/1 -> Data Store Write53/1
  algo_maxClimbSpeed/1 -> Data Store Write22/1
  algo_mode/1 -> Data Type Conversion18/1
  algo_remote_ct_st_yaw/1 -> Data Store Write58/1
  algo_prePathPoint_LLA_0/1 -> Data Store Write25/1
  gy_f2/1 -> Gain91/1
  gz_f2/1 -> Gain92/1
  gx_f2/1 -> Gain41/1
  ax_f/1 -> Data Store Write13/1
  Gain41/1 -> Data Store Write13/4
  az_f/1 -> Data Store Write13/3
  Gain91/1 -> Data Store Write13/5
  ay_f/1 -> Data Store Write13/2
  Gain92/1 -> Data Store Write13/6
  yaw_t/1 -> Data Store Write7/3
  roll_t/1 -> Data Store Write7/1
  pitch_t/1 -> Data Store Write7/2
  algo_curr_vel_0/1 -> Data Store Write28/1
  algo_curr_vel_1/1 -> Data Store Write28/2
  algo_curr_vel_2/1 -> Data Store Write28/3
  Clock2/1 -> algo_maxClimbSpeed/1, algo_flightTaskMode/1, algo_flightControlMode/1, algo_heightCmd/1, algo_turnCenterLL_1/1, algo_prePathPoint_LLA_1/1, algo_prePathPoint_LLA_0/1, algo_rollCmd/1, EAS2TAS_Algo/1, algo_curr_vel_2/1, algo_curr_vel_1/1, algo_curr_vel_0/1, pitch_t/1, roll_t/1, gx_f2/1, az_f/1, ax_f/1, algo_plane_mode/1, Data Store Write5/1, ay_f/1, gy_f2/1, gz_f2/1, yaw_t/1, algo_curr_alt/1, algo_current_loc_0/1, algo_current_loc_1/1, EAS_Algo1/1, algo_mode/1, algo_remote_ct_st_throttle/1, algo_remote_ct_st_pitch/1, algo_remote_ct_st_roll/1, algo_remote_ct_st_yaw/1, algo_curPathPoint_LLA_0/1, algo_curPathPoint_LLA_1/1, algo_turnCenterLL_0/1
  algo_current_loc_0/1 -> Data Store Write8/2
  algo_curr_alt/1 -> Data Store Write8/1
  algo_current_loc_1/1 -> Data Store Write29/1
  EAS_Algo1/1 -> Data Store Write9/1
  EAS2TAS_Algo/1 -> Data Store Write11/1
  Gain147/1 -> Data Store Write34/1
  Gain137/1 -> Data Store Write37/1
  Gain148/1 -> Data Store Write33/1
  Gain164/1 -> Data Store Write64/1
  Clock1/1 -> algo_k_aileron/1, algo_k_rudder/1, algo_latAccDem/1, algo_throttle_dem/1, algo_pitch_dem/1, algo_nav_roll/1, algo_nav_pitch_cd/1, algo_arspeed/1, algo_tail_tilt/1, algo_pwm_out_3/1, algo_pwm_out_2/1, algo_pwm_out_1/1, algo_throttle_filter/1, algo_throttle_in/1, algo_yaw_in/1, algo_pitch_in/1, algo_roll_in/1, algo_rate_target_ang_vel_2/1, algo_rate_target_ang_vel_1/1, algo_rate_target_ang_vel_0/1, algo_attitude_target_euler_rate_2/1, algo_attitude_target_euler_rate_1/1, algo_attitude_target_euler_rate_0/1, algo_attitude_target_euler_angle_2/1, algo_attitude_target_euler_angle_1/1, algo_attitude_target_euler_angle_0/1, algo_climb_rate_cms/1, algo_accel_target_2/1, algo_accel_target_1/1, algo_accel_target_0/1, algo_vel_desired_2/1, algo_vel_target_2/1, algo_vel_target_1/1, algo_vel_target_0/1, algo_curr_pos_0/1, algo_pos_target_2/1, algo_pos_target_1/1, algo_pos_target_0/1, algo_throttle_upper/1, algo_limit_pos_up/1, algo_throttle_lower/1, algo_curr_pos_1/1, algo_z_accel_meas/1, algo_weathervane_last_output/1, algo_pwm_out_4/1, algo_hgt_dem/1, algo_curVelNED_1/1, algo_curVelNED_0/1, algo_curPosNED_1/1, algo_curPosNED_0/1, algo_roll_target_pilot/1, algo_pitch_target_pilot/1, algo_k_throttle/1, algo_k_elevator/1
  algo_pos_target_0/1 -> Scope11/1
  algo_pos_target_1/1 -> Scope12/1
  algo_pos_target_2/1 -> Scope13/1
  Data Store Read12/1 -> Scope11/2
  Data Store Read13/1 -> Scope12/2
  Data Store Read16/1 -> Scope13/2
  Data Store Read17/1 -> Scope14/2
  algo_curr_pos_0/1 -> Scope14/1
  algo_curr_pos_1/1 -> Scope25/1
  Data Store Read20/1 -> Scope25/2
  Data Store Read33/1 -> Scope40/2
  algo_vel_target_1/1 -> Scope40/1
  algo_vel_target_0/1 -> Scope28/1
  Data Store Read32/1 -> Scope28/2
  algo_vel_target_2/1 -> Scope41/1
  Data Store Read34/1 -> Scope41/2
  Data Store Read35/1 -> Scope42/2
  algo_vel_desired_2/1 -> Scope42/1
  algo_accel_target_0/1 -> Scope43/1
  Data Store Read36/1 -> Scope43/2
  Data Store Read37/1 -> Scope44/2
  algo_accel_target_1/1 -> Scope44/1
  algo_accel_target_2/1 -> Scope45/1
  Data Store Read38/1 -> Scope45/2
  Data Store Read39/1 -> Scope46/2
  algo_z_accel_meas/1 -> Scope46/1
  algo_climb_rate_cms/1 -> Scope47/1
  Data Store Read40/1 -> Scope47/2
  Data Store Read41/1 -> Scope48/2
  algo_attitude_target_euler_angle_0/1 -> Scope48/1
  algo_attitude_target_euler_angle_1/1 -> Scope49/1
  Data Store Read42/1 -> Scope49/2
  Data Store Read43/1 -> Scope50/2
  algo_attitude_target_euler_angle_2/1 -> Scope50/1
  algo_attitude_target_euler_rate_0/1 -> Scope51/1
  Data Store Read44/1 -> Scope51/2
  Data Store Read45/1 -> Scope54/2
  algo_attitude_target_euler_rate_1/1 -> Scope54/1
  algo_attitude_target_euler_rate_2/1 -> Scope55/1
  Data Store Read46/1 -> Scope55/2
  Data Store Read48/1 -> Scope56/2
  algo_rate_target_ang_vel_0/1 -> Scope56/1
  algo_rate_target_ang_vel_1/1 -> Scope57/1
  Data Store Read50/1 -> Scope57/2
  Data Store Read51/1 -> Scope58/2
  algo_rate_target_ang_vel_2/1 -> Scope58/1
  algo_roll_in/1 -> Scope59/1
  Data Store Read52/1 -> Scope59/2
  Data Store Read53/1 -> Scope60/2
  algo_pitch_in/1 -> Scope60/1
  algo_yaw_in/1 -> Scope61/1
  Data Store Read54/1 -> Scope61/2
  Data Store Read55/1 -> Scope62/2
  algo_throttle_in/1 -> Scope62/1
  algo_throttle_filter/1 -> Scope63/1
  Data Store Read58/1 -> Scope63/2
  Data Store Read59/1 -> Scope64/2
  algo_weathervane_last_output/1 -> Scope64/1
  algo_pwm_out_1/1 -> Scope69/1
  Data Store Read61/1 -> Scope69/2
  Data Store Read65/1 -> Scope70/2
  algo_pwm_out_2/1 -> Scope70/1
  algo_pwm_out_3/1 -> Scope72/1
  Data Store Read66/1 -> Scope72/2
  Data Store Read67/1 -> Scope73/2
  algo_pwm_out_4/1 -> Scope73/1
  algo_tail_tilt/1 -> Scope74/1
  Data Store Read69/1 -> Scope74/2
  Data Store Read72/1 -> Scope75/2
  algo_arspeed/1 -> Scope75/1
  algo_nav_pitch_cd/1 -> Scope80/1
  Data Store Read73/1 -> Scope80/2
  Data Store Read77/1 -> Scope81/2
  algo_nav_roll/1 -> Scope81/1
  algo_pitch_dem/1 -> Scope83/1
  Data Store Read78/1 -> Scope83/2
  Data Store Read79/1 -> Scope84/2
  algo_throttle_dem/1 -> Scope84/1
  algo_latAccDem/1 -> Scope85/1
  Data Store Read80/1 -> Scope85/2
  Data Store Read81/1 -> Scope87/2
  algo_k_rudder/1 -> Scope87/1
  algo_k_aileron/1 -> Scope88/1
  Data Store Read83/1 -> Scope88/2
  Data Store Read84/1 -> Scope96/2
  algo_k_elevator/1 -> Scope96/1
  algo_k_throttle/1 -> Scope98/1
  Data Store Read85/1 -> Scope98/2
  Data Type Conversion18/1 -> Scope99/1, Data Store Write40/1
  Data Store Read86/1 -> Scope102/1
